simulink model "LowLevel_Example"  (R2024a)
settings: Solver=VariableStepAuto  StartTime=0.0  StopTime=10.0  RelTol=1e-3
model workspace (MAT data in the model file):
  Var = 0
  architecture_gsCommands = Simulink.Bus
  architecture_gsCommands.Alignment = -1
  architecture_gsCommands.PreserveElementDimensions = 0
  architecture_gsCommands.Elements_internal(1) = Simulink.BusElement
  architecture_gsCommands.Elements_internal(1).DimensionsMode = 'Fixed'
  architecture_gsCommands.Elements_internal(1).SamplingMode = 'Sample based'
  architecture_gsCommands.Elements_internal(1).SampleTime = -1
  architecture_gsCommands.Elements_internal(1).Name = 'apConfigParams'
  architecture_gsCommands.Elements_internal(1).DataType_internal = 'Bus: param_value_bus'
  architecture_gsCommands.Elements_internal(1).Complexity = 'real'
  architecture_gsCommands.Elements_internal(1).Dimensions = 1
  architecture_gsCommands.Elements_internal(2) = Simulink.BusElement
  architecture_gsCommands.Elements_internal(2).DimensionsMode = 'Fixed'
  architecture_gsCommands.Elements_internal(2).SamplingMode = 'Sample based'
  architecture_gsCommands.Elements_internal(2).SampleTime = -1
  architecture_gsCommands.Elements_internal(2).Name = 'gsCommands'
  architecture_gsCommands.Elements_internal(2).DataType_internal = 'Bus: gs_commands_bus'
  architecture_gsCommands.Elements_internal(2).Complexity = 'real'
  architecture_gsCommands.Elements_internal(2).Dimensions = 1
  architecture_gsCommands.Elements_internal(3) = Simulink.BusElement
  architecture_gsCommands.Elements_internal(3).DimensionsMode = 'Fixed'
  architecture_gsCommands.Elements_internal(3).SamplingMode = 'Sample based'
  architecture_gsCommands.Elements_internal(3).SampleTime = -1
  architecture_gsCommands.Elements_internal(3).Name = 'uavMission'
  architecture_gsCommands.Elements_internal(3).DataType_internal = 'Bus: mission_item_bus'
  architecture_gsCommands.Elements_internal(3).Complexity = 'real'
  architecture_gsCommands.Elements_internal(3).Dimensions = 1
  architecture_gsCommands.DataScope = 'Auto'
  ctrlSrfcDeflection = Simulink.Bus
  ctrlSrfcDeflection.Alignment = -1
  ctrlSrfcDeflection.PreserveElementDimensions = 0
  ctrlSrfcDeflection.Elements_internal(1) = Simulink.BusElement
  ctrlSrfcDeflection.Elements_internal(1).DimensionsMode = 'Fixed'
  ctrlSrfcDeflection.Elements_internal(1).SamplingMode = 'Sample based'
  ctrlSrfcDeflection.Elements_internal(1).SampleTime = -1
  ctrlSrfcDeflection.Elements_internal(1).Name = 'dA_dF'
  ctrlSrfcDeflection.Elements_internal(1).DataType_internal = 'double'
  ctrlSrfcDeflection.Elements_internal(1).Complexity = 'real'
  ctrlSrfcDeflection.Elements_internal(1).Dimensions = 1
  ctrlSrfcDeflection.Elements_internal(2) = Simulink.BusElement
  ctrlSrfcDeflection.Elements_internal(2).DimensionsMode = 'Fixed'
  ctrlSrfcDeflection.Elements_internal(2).SamplingMode = 'Sample based'
  ctrlSrfcDeflection.Elements_internal(2).SampleTime = -1
  ctrlSrfcDeflection.Elements_internal(2).Name = 'Brake'
  ctrlSrfcDeflection.Elements_internal(2).DataType_internal = 'double'
  ctrlSrfcDeflection.Elements_internal(2).Complexity = 'real'
  ctrlSrfcDeflection.Elements_internal(2).Dimensions = 1
  ctrlSrfcDeflection.Elements_internal(3) = Simulink.BusElement
  ctrlSrfcDeflection.Elements_internal(3).DimensionsMode = 'Fixed'
  ctrlSrfcDeflection.Elements_internal(3).SamplingMode = 'Sample based'
  ctrlSrfcDeflection.Elements_internal(3).SampleTime = -1
  ctrlSrfcDeflection.Elements_internal(3).Name = 'dR_dE'
  ctrlSrfcDeflection.Elements_internal(3).DataType_internal = 'double'
  ctrlSrfcDeflection.Elements_internal(3).Complexity = 'real'
  ctrlSrfcDeflection.Elements_internal(3).Dimensions = 1
  ctrlSrfcDeflection.DataScope = 'Auto'
  gs_commands_bus = Simulink.Bus
  gs_commands_bus.Alignment = -1
  gs_commands_bus.PreserveElementDimensions = 0
  gs_commands_bus.Elements_internal(1) = Simulink.BusElement
  gs_commands_bus.Elements_internal(1).DimensionsMode = 'Fixed'
  gs_commands_bus.Elements_internal(1).SamplingMode = 'Sample based'
  gs_commands_bus.Elements_internal(1).SampleTime = -1
  gs_commands_bus.Elements_internal(1).Description = 'Return to Base Command'
  gs_commands_bus.Elements_internal(1).Name = 'RTB'
  gs_commands_bus.Elements_internal(1).DataType_internal = 'uint8'
  gs_commands_bus.Elements_internal(1).Complexity = 'real'
  gs_commands_bus.Elements_internal(1).Dimensions = 1
  gs_commands_bus.Elements_internal(2) = Simulink.BusElement
  gs_commands_bus.Elements_internal(2).DimensionsMode = 'Fixed'
  gs_commands_bus.Elements_internal(2).SamplingMode = 'Sample based'
  gs_commands_bus.Elements_internal(2).SampleTime = -1
  gs_commands_bus.Elements_internal(2).Description = 'Airspeed Commanded by the GS'
  gs_commands_bus.Elements_internal(2).Name = 'U_c'
  gs_commands_bus.Elements_internal(2).DataType_internal = 'single'
  gs_commands_bus.Elements_internal(2).Complexity = 'real'
  gs_commands_bus.Elements_internal(2).Dimensions = 1
  gs_commands_bus.Elements_internal(3) = Simulink.BusElement
  gs_commands_bus.Elements_internal(3).DimensionsMode = 'Fixed'
  gs_commands_bus.Elements_internal(3).SamplingMode = 'Sample based'
  gs_commands_bus.Elements_internal(3).SampleTime = -1
  gs_commands_bus.Elements_internal(3).Description = 'Turnrate command when in mid Level Commands guidance mode'
  gs_commands_bus.Elements_internal(3).Name = 'psiDot_c_mdiLevel'
  gs_commands_bus.Elements_internal(3).DataType_internal = 'single'
  gs_commands_bus.Elements_internal(3).Complexity = 'real'
  gs_commands_bus.Elements_internal(3).Dimensions = 1
  gs_commands_bus.Elements_internal(4) = Simulink.BusElement
  gs_commands_bus.Elements_internal(4).DimensionsMode = 'Fixed'
  gs_commands_bus.Elements_internal(4).SamplingMode = 'Sample based'
  gs_commands_bus.Elements_internal(4).SampleTime = -1
  gs_commands_bus.Elements_internal(4).Description = 'Commanded altitude when in Mid Level Commands Mode. Also used as the altitude for RTB'
  gs_commands_bus.Elements_internal(4).Name = 'h_c_midLevel'
  gs_commands_bus.Elements_internal(4).DataType_internal = 'single'
  gs_commands_bus.Elements_internal(4).Complexity = 'real'
  gs_commands_bus.Elements_internal(4).Dimensions = 1
  gs_commands_bus.Elements_internal(5) = Simulink.BusElement
  gs_commands_bus.Elements_internal(5).DimensionsMode = 'Fixed'
  gs_commands_bus.Elements_internal(5).SamplingMode = 'Sample based'
  gs_commands_bus.Elements_internal(5).SampleTime = -1
  gs_commands_bus.Elements_internal(5).Name = 'isManualModeOn'
  gs_commands_bus.Elements_internal(5).DataType_internal = 'uint8'
  gs_commands_bus.Elements_internal(5).Complexity = 'real'
  gs_commands_bus.Elements_internal(5).Dimensions = 1
  gs_commands_bus.Elements_internal(6) = Simulink.BusElement
  gs_commands_bus.Elements_internal(6).DimensionsMode = 'Fixed'
  gs_commands_bus.Elements_internal(6).SamplingMode = 'Sample based'
  gs_commands_bus.Elements_internal(6).SampleTime = -1
  gs_commands_bus.Elements_internal(6).Name = 'viewPointIdx'
  gs_commands_bus.Elements_internal(6).DataType_internal = 'uint8'
  gs_commands_bus.Elements_internal(6).Complexity = 'real'
  gs_commands_bus.Elements_internal(6).Dimensions = 1
  gs_commands_bus.Elements_internal(7) = Simulink.BusElement
  gs_commands_bus.Elements_internal(7).DimensionsMode = 'Fixed'
  gs_commands_bus.Elements_internal(7).SamplingMode = 'Sample based'
  gs_commands_bus.Elements_internal(7).SampleTime = -1
  gs_commands_bus.Elements_internal(7).Name = 'guidanceMode'
  gs_commands_bus.Elements_internal(7).DataType_internal = 'uint8'
  gs_commands_bus.Elements_internal(7).Complexity = 'real'
  gs_commands_bus.Elements_internal(7).Dimensions = 1
  gs_commands_bus.DataScope = 'Auto'
  lightCmds = Simulink.Bus
  lightCmds.Alignment = -1
  lightCmds.PreserveElementDimensions = 0
  lightCmds.Elements_internal(1) = Simulink.BusElement
  lightCmds.Elements_internal(1).DimensionsMode = 'Fixed'
  lightCmds.Elements_internal(1).SamplingMode = 'Sample based'
  lightCmds.Elements_internal(1).SampleTime = -1
  lightCmds.Elements_internal(1).Name = 'NavigationLights'
  lightCmds.Elements_internal(1).DataType_internal = 'double'
  lightCmds.Elements_internal(1).Complexity = 'real'
  lightCmds.Elements_internal(1).Dimensions = 1
  lightCmds.Elements_internal(2) = Simulink.BusElement
  lightCmds.Elements_internal(2).DimensionsMode = 'Fixed'
  lightCmds.Elements_internal(2).SamplingMode = 'Sample based'
  lightCmds.Elements_internal(2).SampleTime = -1
  lightCmds.Elements_internal(2).Name = 'LandingStrobe'
  lightCmds.Elements_internal(2).DataType_internal = 'double'
  lightCmds.Elements_internal(2).Complexity = 'real'
  lightCmds.Elements_internal(2).Dimensions = 1
  lightCmds.DataScope = 'Auto'
  mission_item_bus = Simulink.Bus
  mission_item_bus.Alignment = -1
  mission_item_bus.PreserveElementDimensions = 0
  mission_item_bus.Elements_internal(1) = Simulink.BusElement
  mission_item_bus.Elements_internal(1).DimensionsMode = 'Fixed'
  mission_item_bus.Elements_internal(1).SamplingMode = 'Sample based'
  mission_item_bus.Elements_internal(1).SampleTime = -1
  mission_item_bus.Elements_internal(1).Description = 'PARAM1, see MAV_CMD enum'
  mission_item_bus.Elements_internal(1).Name = 'param1'
  mission_item_bus.Elements_internal(1).DataType_internal = 'single'
  mission_item_bus.Elements_internal(1).Complexity = 'real'
  mission_item_bus.Elements_internal(1).Dimensions = 1
  mission_item_bus.Elements_internal(2) = Simulink.BusElement
  mission_item_bus.Elements_internal(2).DimensionsMode = 'Fixed'
  mission_item_bus.Elements_internal(2).SamplingMode = 'Sample based'
  mission_item_bus.Elements_internal(2).SampleTime = -1
  mission_item_bus.Elements_internal(2).Description = 'PARAM4, see MAV_CMD enum'
  mission_item_bus.Elements_internal(2).Name = 'param4'
  mission_item_bus.Elements_internal(2).DataType_internal = 'single'
  mission_item_bus.Elements_internal(2).Complexity = 'real'
  mission_item_bus.Elements_internal(2).Dimensions = 1
  mission_item_bus.Elements_internal(3) = Simulink.BusElement
  mission_item_bus.Elements_internal(3).DimensionsMode = 'Fixed'
  mission_item_bus.Elements_internal(3).SamplingMode = 'Sample based'
  mission_item_bus.Elements_internal(3).SampleTime = -1
  mission_item_bus.Elements_internal(3).Description = 'PARAM3, see MAV_CMD enum'
  mission_item_bus.Elements_internal(3).Name = 'param3'
  mission_item_bus.Elements_internal(3).DataType_internal = 'single'
  mission_item_bus.Elements_internal(3).Complexity = 'real'
  mission_item_bus.Elements_internal(3).Dimensions = 1
  mission_item_bus.Elements_internal(4) = Simulink.BusElement
  mission_item_bus.Elements_internal(4).DimensionsMode = 'Fixed'
  mission_item_bus.Elements_internal(4).SamplingMode = 'Sample based'
  mission_item_bus.Elements_internal(4).SampleTime = -1
  mission_item_bus.Elements_internal(4).Description = 'false:0, true:1'
  mission_item_bus.Elements_internal(4).Name = 'current'
  mission_item_bus.Elements_internal(4).DataType_internal = 'uint8'
  mission_item_bus.Elements_internal(4).Complexity = 'real'
  mission_item_bus.Elements_internal(4).Dimensions = 1
  mission_item_bus.Elements_internal(5) = Simulink.BusElement
  mission_item_bus.Elements_internal(5).DimensionsMode = 'Fixed'
  mission_item_bus.Elements_internal(5).SamplingMode = 'Sample based'
  mission_item_bus.Elements_internal(5).SampleTime = -1
  mission_item_bus.Elements_internal(5).Description = 'PARAM2, see MAV_CMD enum'
  mission_item_bus.Elements_internal(5).Name = 'param2'
  mission_item_bus.Elements_internal(5).DataType_internal = 'single'
  mission_item_bus.Elements_internal(5).Complexity = 'real'
  mission_item_bus.Elements_internal(5).Dimensions = 1
  mission_item_bus.Elements_internal(6) = Simulink.BusElement
  mission_item_bus.Elements_internal(6).DimensionsMode = 'Fixed'
  mission_item_bus.Elements_internal(6).SamplingMode = 'Sample based'
  mission_item_bus.Elements_internal(6).SampleTime = -1
  mission_item_bus.Elements_internal(6).Description = 'PARAM5 / local: x position, global: latitude'
  mission_item_bus.Elements_internal(6).Name = 'x'
  mission_item_bus.Elements_internal(6).DataType_internal = 'single'
  mission_item_bus.Elements_internal(6).Complexity = 'real'
  mission_item_bus.Elements_internal(6).Dimensions = 1
  mission_item_bus.Elements_internal(7) = Simulink.BusElement
  mission_item_bus.Elements_internal(7).DimensionsMode = 'Fixed'
  mission_item_bus.Elements_internal(7).SamplingMode = 'Sample based'
  mission_item_bus.Elements_internal(7).SampleTime = -1
  mission_item_bus.Elements_internal(7).Description = 'PARAM6 / y position: global: longitude'
  mission_item_bus.Elements_internal(7).Name = 'y'
  mission_item_bus.Elements_internal(7).DataType_internal = 'single'
  mission_item_bus.Elements_internal(7).Complexity = 'real'
  mission_item_bus.Elements_internal(7).Dimensions = 1
  mission_item_bus.Elements_internal(8) = Simulink.BusElement
  mission_item_bus.Elements_internal(8).DimensionsMode = 'Fixed'
  mission_item_bus.Elements_internal(8).SamplingMode = 'Sample based'
  mission_item_bus.Elements_internal(8).SampleTime = -1
  mission_item_bus.Elements_internal(8).Description = 'The scheduled action for the waypoint. see MAV_CMD in common.xml MAVLink specs'
  mission_item_bus.Elements_internal(8).Name = 'command'
  mission_item_bus.Elements_internal(8).DataType_internal = 'uint16'
  mission_item_bus.Elements_internal(8).Complexity = 'real'
  mission_item_bus.Elements_internal(8).Dimensions = 1
  mission_item_bus.Elements_internal(9) = Simulink.BusElement
  mission_item_bus.Elements_internal(9).DimensionsMode = 'Fixed'
  mission_item_bus.Elements_internal(9).SamplingMode = 'Sample based'
  mission_item_bus.Elements_internal(9).SampleTime = -1
  mission_item_bus.Elements_internal(9).Description = 'PARAM7 / z position: global: altitude (relative or absolute, depending on frame.'
  mission_item_bus.Elements_internal(9).Name = 'z'
  mission_item_bus.Elements_internal(9).DataType_internal = 'single'
  mission_item_bus.Elements_internal(9).Complexity = 'real'
  mission_item_bus.Elements_internal(9).Dimensions = 1
  mission_item_bus.Elements_internal(10) = Simulink.BusElement
  mission_item_bus.Elements_internal(10).DimensionsMode = 'Fixed'
  mission_item_bus.Elements_internal(10).SamplingMode = 'Sample based'
  mission_item_bus.Elements_internal(10).SampleTime = -1
  mission_item_bus.Elements_internal(10).Description = 'System ID'
  mission_item_bus.Elements_internal(10).Name = 'target_system'
  mission_item_bus.Elements_internal(10).DataType_internal = 'uint8'
  mission_item_bus.Elements_internal(10).Complexity = 'real'
  mission_item_bus.Elements_internal(10).Dimensions = 1
  mission_item_bus.Elements_internal(11) = Simulink.BusElement
  mission_item_bus.Elements_internal(11).DimensionsMode = 'Fixed'
  mission_item_bus.Elements_internal(11).SamplingMode = 'Sample based'
  mission_item_bus.Elements_internal(11).SampleTime = -1
  mission_item_bus.Elements_internal(11).Description = 'Sequence'
  mission_item_bus.Elements_internal(11).Name = 'seq'
  mission_item_bus.Elements_internal(11).DataType_internal = 'uint16'
  mission_item_bus.Elements_internal(11).Complexity = 'real'
  mission_item_bus.Elements_internal(11).Dimensions = 1
  mission_item_bus.Elements_internal(12) = Simulink.BusElement
  mission_item_bus.Elements_internal(12).DimensionsMode = 'Fixed'
  mission_item_bus.Elements_internal(12).SamplingMode = 'Sample based'
  mission_item_bus.Elements_internal(12).SampleTime = -1
  mission_item_bus.Elements_internal(12).Description = 'Mission type, see MAV_MISSION_TYPE'
  mission_item_bus.Elements_internal(12).Name = 'mission_type'
  mission_item_bus.Elements_internal(12).DataType_internal = 'uint8'
  mission_item_bus.Elements_internal(12).Complexity = 'real'
  mission_item_bus.Elements_internal(12).Dimensions = 1
  mission_item_bus.Elements_internal(13) = Simulink.BusElement
  mission_item_bus.Elements_internal(13).DimensionsMode = 'Fixed'
  mission_item_bus.Elements_internal(13).SamplingMode = 'Sample based'
  mission_item_bus.Elements_internal(13).SampleTime = -1
  mission_item_bus.Elements_internal(13).Description = 'The coordinate system of the waypoint. see MAV_FRAME in mavlink_types.h'
  mission_item_bus.Elements_internal(13).Name = 'frame'
  mission_item_bus.Elements_internal(13).DataType_internal = 'uint8'
  mission_item_bus.Elements_internal(13).Complexity = 'real'
  mission_item_bus.Elements_internal(13).Dimensions = 1
  mission_item_bus.Elements_internal(14) = Simulink.BusElement
  mission_item_bus.Elements_internal(14).DimensionsMode = 'Fixed'
  mission_item_bus.Elements_internal(14).SamplingMode = 'Sample based'
  mission_item_bus.Elements_internal(14).SampleTime = -1
  mission_item_bus.Elements_internal(14).Description = 'Component ID'
  mission_item_bus.Elements_internal(14).Name = 'target_component'
  mission_item_bus.Elements_internal(14).DataType_internal = 'uint8'
  mission_item_bus.Elements_internal(14).Complexity = 'real'
  mission_item_bus.Elements_internal(14).Dimensions = 1
  mission_item_bus.Elements_internal(15) = Simulink.BusElement
  mission_item_bus.Elements_internal(15).DimensionsMode = 'Fixed'
  mission_item_bus.Elements_internal(15).SamplingMode = 'Sample based'
  mission_item_bus.Elements_internal(15).SampleTime = -1
  mission_item_bus.Elements_internal(15).Description = 'autocontinue to next wp'
  mission_item_bus.Elements_internal(15).Name = 'autocontinue'
  mission_item_bus.Elements_internal(15).DataType_internal = 'uint8'
  mission_item_bus.Elements_internal(15).Complexity = 'real'
  mission_item_bus.Elements_internal(15).Dimensions = 1
  mission_item_bus.DataScope = 'Auto'
  operatorCmds = Simulink.Bus
  operatorCmds.Alignment = -1
  operatorCmds.PreserveElementDimensions = 0
  operatorCmds.Elements_internal(1) = Simulink.BusElement
  operatorCmds.Elements_internal(1).DimensionsMode = 'Fixed'
  operatorCmds.Elements_internal(1).SamplingMode = 'Sample based'
  operatorCmds.Elements_internal(1).SampleTime = -1
  operatorCmds.Elements_internal(1).Name = 'RetractorCmds'
  operatorCmds.Elements_internal(1).DataType_internal = 'double'
  operatorCmds.Elements_internal(1).Complexity = 'real'
  operatorCmds.Elements_internal(1).Dimensions = 1
  operatorCmds.Elements_internal(2) = Simulink.BusElement
  operatorCmds.Elements_internal(2).DimensionsMode = 'Fixed'
  operatorCmds.Elements_internal(2).SamplingMode = 'Sample based'
  operatorCmds.Elements_internal(2).SampleTime = -1
  operatorCmds.Elements_internal(2).Name = 'PTZCmds'
  operatorCmds.Elements_internal(2).DataType_internal = 'double'
  operatorCmds.Elements_internal(2).Complexity = 'real'
  operatorCmds.Elements_internal(2).Dimensions = 1
  operatorCmds.DataScope = 'Auto'
  param_value_bus = Simulink.Bus
  param_value_bus.Alignment = -1
  param_value_bus.PreserveElementDimensions = 0
  param_value_bus.Elements_internal(1) = Simulink.BusElement
  param_value_bus.Elements_internal(1).DimensionsMode = 'Fixed'
  param_value_bus.Elements_internal(1).SamplingMode = 'Sample based'
  param_value_bus.Elements_internal(1).SampleTime = -1
  param_value_bus.Elements_internal(1).Description = 'Onboard parameter value'
  param_value_bus.Elements_internal(1).Name = 'param_value'
  param_value_bus.Elements_internal(1).DataType_internal = 'single'
  param_value_bus.Elements_internal(1).Complexity = 'real'
  param_value_bus.Elements_internal(1).Dimensions = 1
  param_value_bus.Elements_internal(2) = Simulink.BusElement
  param_value_bus.Elements_internal(2).DimensionsMode = 'Fixed'
  param_value_bus.Elements_internal(2).SamplingMode = 'Sample based'
  param_value_bus.Elements_internal(2).SampleTime = -1
  param_value_bus.Elements_internal(2).Description = 'Index of this onboard parameter'
  param_value_bus.Elements_internal(2).Name = 'param_index'
  param_value_bus.Elements_internal(2).DataType_internal = 'uint16'
  param_value_bus.Elements_internal(2).Complexity = 'real'
  param_value_bus.Elements_internal(2).Dimensions = 1
  param_value_bus.Elements_internal(3) = Simulink.BusElement
  param_value_bus.Elements_internal(3).DimensionsMode = 'Fixed'
  param_value_bus.Elements_internal(3).SamplingMode = 'Sample based'
  param_value_bus.Elements_internal(3).SampleTime = -1
  param_value_bus.Elements_internal(3).Description = 'Total number of onboard parameters'
  param_value_bus.Elements_internal(3).Name = 'param_count'
  param_value_bus.Elements_internal(3).DataType_internal = 'uint16'
  param_value_bus.Elements_internal(3).Complexity = 'real'
  param_value_bus.Elements_internal(3).Dimensions = 1
  param_value_bus.Elements_internal(4) = Simulink.BusElement
  param_value_bus.Elements_internal(4).DimensionsMode = 'Fixed'
  param_value_bus.Elements_internal(4).SamplingMode = 'Sample based'
  param_value_bus.Elements_internal(4).SampleTime = -1
  param_value_bus.Elements_internal(4).Description = 'Onboard parameter id, terminated by NULL if the length is less than 16 human-readable chars and WITHOUT null termination (NULL) byte if the length is exactly 16 chars - applications have to provide 16+1 bytes storage if the ID is stored as string'
  param_value_bus.Elements_internal(4).Name = 'param_id'
  param_value_bus.Elements_internal(4).DataType_internal = 'int8'
  param_value_bus.Elements_internal(4).Complexity = 'real'
  param_value_bus.Elements_internal(4).Dimensions = 16
  param_value_bus.Elements_internal(5) = Simulink.BusElement
  param_value_bus.Elements_internal(5).DimensionsMode = 'Fixed'
  param_value_bus.Elements_internal(5).SamplingMode = 'Sample based'
  param_value_bus.Elements_internal(5).SampleTime = -1
  param_value_bus.Elements_internal(5).Description = 'Onboard parameter type: see the MAV_PARAM_TYPE enum for supported data types.'
  param_value_bus.Elements_internal(5).Name = 'param_type'
  param_value_bus.Elements_internal(5).DataType_internal = 'uint8'
  param_value_bus.Elements_internal(5).Complexity = 'real'
  param_value_bus.Elements_internal(5).Dimensions = 1
  param_value_bus.DataScope = 'Auto'
(part 1 of 2)
settings Model: Creator=The MathWorks, Inc.  LastModifiedBy=Tamir Azaouag
settings SolverCC: AlgebraicLoopSolver=TrustRegion
settings DebuggingCC: UnconnectedLineMsg=warning
settings ModelReferenceCC: EnableRefExpFcnMdlSchedulingChecks=on
settings RTWCC: GPUComputeCapability=3.5  DLArmComputeVersion=19.05

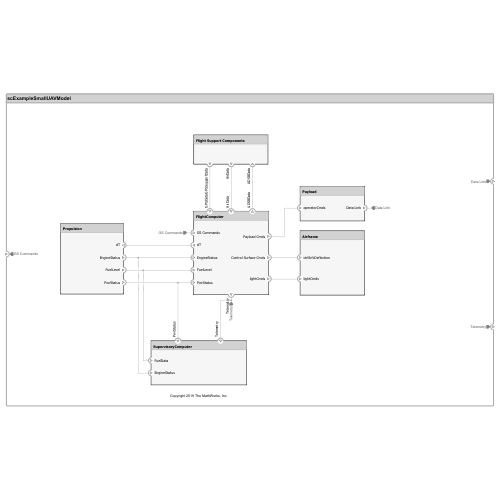
[thumbnail: Simulink's stored preview of the top-level diagram]
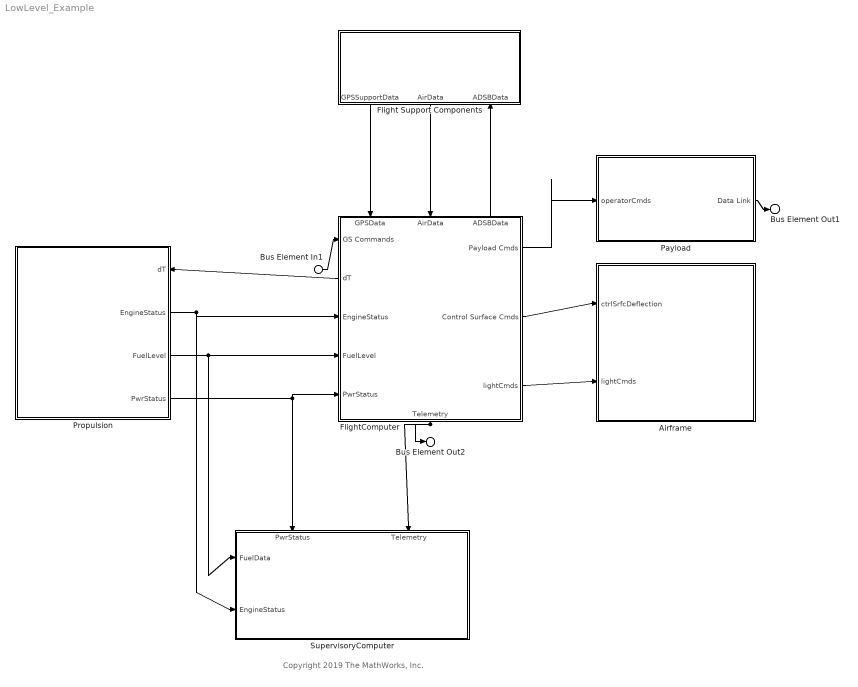
== system LowLevel_Example ==
  note: Copyright 2019 The MathWorks, Inc.
  Bus Element In1 : Inport  PortName=GS Commands
  Airframe : Subsystem
      settings: PortSchema="{\"entries\":[{\"content\":{\"headerSize\":26,\"margin\":15,\"minimumSpacing\":25,\"sides\":[{\"content\":{\"connectorIds\":[\"In1\",\"In2\"]},\"type\":\"ConnectorPlacement.EquallySpacedRectSide\",\"uuid\":\"410c5b0f-08b5-48c1-aeab-ad32707f18cb\"},{\"content\":{\"connectorIds\":[],\"side\":\"RIGHT\"},\"type\":\"ConnectorPlacement.EquallySpacedRectSide\",\"uuid\":\"175f376c-06cb-43d8-93cf-cfe74288c6ca\"},{\"content\":{\"connectorIds\":[],\"side\":\"TOP\"},\"type\":\"ConnectorPlacement.EquallySpacedRectSide\",\"uuid\":\"49daa1ce-2b00-43ab-833d-e4aa679275fe\"}]},\"type\":\"ConnectorPlacement.EquallySpacedConnector\",\"uuid\":\"5fe6ec80-a25e-4dcf-8012-d525fb653d3d\"}],\"packageUris\":[\"http:\\/\\/schema.mathworks.com\\/mf0\\/Connector\\/19700101\"],\"version\":\"1.0\"}"
  Flight Support Components : Subsystem
      settings: PortSchema="{\"entries\":[{\"content\":{\"headerSize\":26,\"margin\":15,\"minimumSpacing\":25,\"sides\":[{\"content\":{\"connectorIds\":[]},\"type\":\"ConnectorPlacement.EquallySpacedRectSide\",\"uuid\":\"410c5b0f-08b5-48c1-aeab-ad32707f18cb\"},{\"content\":{\"connectorIds\":[],\"side\":\"RIGHT\"},\"type\":\"ConnectorPlacement.EquallySpacedRectSide\",\"uuid\":\"175f376c-06cb-43d8-93cf-cfe74288c6ca\"},{\"content\":{\"connectorIds\":[],\"side\":\"TOP\"},\"type\":\"ConnectorPlacement.EquallySpacedRectSide\",\"uuid\":\"49daa1ce-2b00-43ab-833d-e4aa679275fe\"},{\"content\":{\"connectorIds\":[\"Out2\",\"Out1\",\"In1\"],\"side\":\"BOTTOM\"},\"type\":\"ConnectorPlacement.EquallySpacedRectSide\",\"uuid\":\"223cc250-646f-4cb8-9a9a-650b4875d99e\"}]},\"type\":\"ConnectorPlacement.EquallySpacedConnector\",\"uuid\":\"5fe6ec80-a25e-4dcf-8012-d525fb653d3d\"}],\"packageUris\":[\"http:\\/\\/schema.mathworks.com\\/mf0\\/Connector\\/19700101\"],\"version\":\"1.0\"}"
  FlightComputer : Subsystem
      settings: PortSchema="{\"entries\":[{\"content\":{\"headerSize\":26,\"margin\":15,\"minimumSpacing\":25,\"sides\":[{\"content\":{\"connectorIds\":[\"In5\",\"Out5\",\"In2\",\"In3\",\"In6\"]},\"type\":\"ConnectorPlacement.EquallySpacedRectSide\",\"uuid\":\"288187f8-f80a-4535-8eff-6998f4e932c0\"},{\"content\":{\"connectorIds\":[\"Out3\",\"Out2\",\"Out6\"],\"side\":\"RIGHT\"},\"type\":\"ConnectorPlacement.EquallySpacedRectSide\",\"uuid\":\"d1e22774-cdd2-4e71-94b1-3e938d9d16f6\"},{\"content\":{\"connectorIds\":[\"In4\",\"In1\",\"Out1\"],\"side\":\"TOP\"},\"type\":\"ConnectorPlacement.EquallySpacedRectSide\",\"uuid\":\"890411bd-a9cd-40b1-a683-0574f0cd14d7\"},{\"content\":{\"connectorIds\":[\"Out4\"],\"side\":\"BOTTOM\"},\"type\":\"ConnectorPlacement.EquallySpacedRectSide\",\"uuid\":\"5b2b87a3-00cb-493f-9187-a9231b1dbd9e\"}]},\"type\":\"ConnectorPlacement.EquallySpacedConnector\",\"uuid\":\"f677e6f7-ddb0-43ad-ab3a-7892dac74d79\"}],\"packageUris\":[\"http:\\/\\/schema.mathworks.com\\/mf0\\/Connector\\/19700101\"],\"version\":\"1.0\"}"
  Payload : Subsystem
      settings: PortSchema="{\"entries\":[{\"content\":{\"headerSize\":26,\"margin\":15,\"minimumSpacing\":25,\"sides\":[{\"content\":{\"connectorIds\":[\"In1\"]},\"type\":\"ConnectorPlacement.EquallySpacedRectSide\",\"uuid\":\"288187f8-f80a-4535-8eff-6998f4e932c0\"},{\"content\":{\"connectorIds\":[\"Out1\"],\"side\":\"RIGHT\"},\"type\":\"ConnectorPlacement.EquallySpacedRectSide\",\"uuid\":\"d1e22774-cdd2-4e71-94b1-3e938d9d16f6\"},{\"content\":{\"connectorIds\":[],\"side\":\"TOP\"},\"type\":\"ConnectorPlacement.EquallySpacedRectSide\",\"uuid\":\"890411bd-a9cd-40b1-a683-0574f0cd14d7\"}]},\"type\":\"ConnectorPlacement.EquallySpacedConnector\",\"uuid\":\"f677e6f7-ddb0-43ad-ab3a-7892dac74d79\"}],\"packageUris\":[\"http:\\/\\/schema.mathworks.com\\/mf0\\/Connector\\/19700101\"],\"version\":\"1.0\"}"
  Propulsion : Subsystem
      settings: PortSchema="{\"entries\":[{\"content\":{\"headerSize\":26,\"margin\":15,\"minimumSpacing\":25,\"sides\":[{\"content\":{\"connectorIds\":[]},\"type\":\"ConnectorPlacement.EquallySpacedRectSide\",\"uuid\":\"288187f8-f80a-4535-8eff-6998f4e932c0\"},{\"content\":{\"connectorIds\":[\"In1\",\"Out1\",\"Out2\",\"Out3\"],\"side\":\"RIGHT\"},\"type\":\"ConnectorPlacement.EquallySpacedRectSide\",\"uuid\":\"d1e22774-cdd2-4e71-94b1-3e938d9d16f6\"},{\"content\":{\"connectorIds\":[],\"side\":\"TOP\"},\"type\":\"ConnectorPlacement.EquallySpacedRectSide\",\"uuid\":\"890411bd-a9cd-40b1-a683-0574f0cd14d7\"}]},\"type\":\"ConnectorPlacement.EquallySpacedConnector\",\"uuid\":\"f677e6f7-ddb0-43ad-ab3a-7892dac74d79\"}],\"packageUris\":[\"http:\\/\\/schema.mathworks.com\\/mf0\\/Connector\\/19700101\"],\"version\":\"1.0\"}"
  SupervisoryComputer : Subsystem
      settings: PortSchema="{\"entries\":[{\"content\":{\"headerSize\":26,\"margin\":15,\"minimumSpacing\":25,\"sides\":[{\"content\":{\"connectorIds\":[\"In2\",\"In1\"]},\"type\":\"ConnectorPlacement.EquallySpacedRectSide\",\"uuid\":\"410c5b0f-08b5-48c1-aeab-ad32707f18cb\"},{\"content\":{\"connectorIds\":[],\"side\":\"RIGHT\"},\"type\":\"ConnectorPlacement.EquallySpacedRectSide\",\"uuid\":\"175f376c-06cb-43d8-93cf-cfe74288c6ca\"},{\"content\":{\"connectorIds\":[\"In3\",\"In4\"],\"side\":\"TOP\"},\"type\":\"ConnectorPlacement.EquallySpacedRectSide\",\"uuid\":\"49daa1ce-2b00-43ab-833d-e4aa679275fe\"}]},\"type\":\"ConnectorPlacement.EquallySpacedConnector\",\"uuid\":\"5fe6ec80-a25e-4dcf-8012-d525fb653d3d\"}],\"packageUris\":[\"http:\\/\\/schema.mathworks.com\\/mf0\\/Connector\\/19700101\"],\"version\":\"1.0\"}"
  Bus Element Out1 : Outport  VectorParamsAs1DForOutWhenUnconnected=off  PortName=Data Link
  Bus Element Out2 : Outport  Port=2  VectorParamsAs1DForOutWhenUnconnected=off  PortName=Telemetry
  wires:
  FlightComputer/1(ADSBData) -> Flight Support Components/1(ADSBData)
  FlightComputer/6(lightCmds) -> Airframe/2(lightCmds)
  Flight Support Components/1(AirData) -> FlightComputer/1(AirData)
  FlightComputer/2(Control Surface Cmds) -> Airframe/1(ctrlSrfcDeflection)
  Flight Support Components/2(GPSSupportData) -> FlightComputer/4(GPSData)
  FlightComputer/5(dT) -> Propulsion/1(dT)
  Payload/1(Data Link) -> Bus Element Out1/1
  FlightComputer/4(Telemetry) -> SupervisoryComputer/4(Telemetry), Bus Element Out2/1
  FlightComputer/3(Payload Cmds) -> Payload/1(operatorCmds)
  Bus Element In1/1 -> FlightComputer/5(GS Commands)
  Propulsion/2(FuelLevel) -> FlightComputer/3(FuelLevel), SupervisoryComputer/2(FuelData)
  Propulsion/3(PwrStatus) -> FlightComputer/6(PwrStatus), SupervisoryComputer/3(PwrStatus)
  Propulsion/1(EngineStatus) -> SupervisoryComputer/1(EngineStatus), FlightComputer/2(EngineStatus)

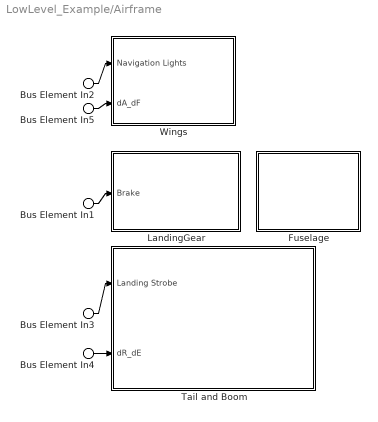
== system LowLevel_Example/Airframe ==
  Bus Element In5 : Inport  PortName=ctrlSrfcDeflection  Element=dA_dF
  Bus Element In1 : Inport  PortName=ctrlSrfcDeflection  Element=Brake
  Bus Element In4 : Inport  PortName=ctrlSrfcDeflection  Element=dR_dE
  Bus Element In2 : Inport  Port=2  PortName=lightCmds  Element=NavigationLights
  Bus Element In3 : Inport  Port=2  PortName=lightCmds  Element=LandingStrobe
  Fuselage : Subsystem
      settings: PortSchema="{\"entries\":[{\"content\":{\"headerSize\":26,\"margin\":15,\"minimumSpacing\":25,\"sides\":[{\"content\":{\"connectorIds\":[]},\"type\":\"ConnectorPlacement.EquallySpacedRectSide\",\"uuid\":\"1d3f3a23-636b-441d-85a6-b75e05b18389\"},{\"content\":{\"connectorIds\":[],\"side\":\"RIGHT\"},\"type\":\"ConnectorPlacement.EquallySpacedRectSide\",\"uuid\":\"e22d7e46-f58c-4c9d-8892-998381cd60e3\"},{\"content\":{\"connectorIds\":[],\"side\":\"TOP\"},\"type\":\"ConnectorPlacement.EquallySpacedRectSide\",\"uuid\":\"8b16ddbb-b471-4974-8372-55ce1efe9f0b\"}]},\"type\":\"ConnectorPlacement.EquallySpacedConnector\",\"uuid\":\"3aaecc83-0a24-4c0b-b096-52d61c24d002\"}],\"packageUris\":[\"http:\\/\\/schema.mathworks.com\\/mf0\\/Connector\\/19700101\"],\"version\":\"1.0\"}"
  LandingGear : Subsystem
      settings: PortSchema="{\"entries\":[{\"content\":{\"headerSize\":26,\"margin\":15,\"minimumSpacing\":25,\"sides\":[{\"content\":{\"connectorIds\":[\"In1\"]},\"type\":\"ConnectorPlacement.EquallySpacedRectSide\",\"uuid\":\"410c5b0f-08b5-48c1-aeab-ad32707f18cb\"},{\"content\":{\"connectorIds\":[],\"side\":\"RIGHT\"},\"type\":\"ConnectorPlacement.EquallySpacedRectSide\",\"uuid\":\"175f376c-06cb-43d8-93cf-cfe74288c6ca\"},{\"content\":{\"connectorIds\":[],\"side\":\"TOP\"},\"type\":\"ConnectorPlacement.EquallySpacedRectSide\",\"uuid\":\"49daa1ce-2b00-43ab-833d-e4aa679275fe\"}]},\"type\":\"ConnectorPlacement.EquallySpacedConnector\",\"uuid\":\"5fe6ec80-a25e-4dcf-8012-d525fb653d3d\"}],\"packageUris\":[\"http:\\/\\/schema.mathworks.com\\/mf0\\/Connector\\/19700101\"],\"version\":\"1.0\"}"
  Tail and Boom : Subsystem
      settings: PortSchema="{\"entries\":[{\"content\":{\"headerSize\":26,\"margin\":15,\"minimumSpacing\":25,\"sides\":[{\"content\":{\"connectorIds\":[\"In1\",\"In2\"]},\"type\":\"ConnectorPlacement.EquallySpacedRectSide\",\"uuid\":\"410c5b0f-08b5-48c1-aeab-ad32707f18cb\"},{\"content\":{\"connectorIds\":[],\"side\":\"RIGHT\"},\"type\":\"ConnectorPlacement.EquallySpacedRectSide\",\"uuid\":\"175f376c-06cb-43d8-93cf-cfe74288c6ca\"},{\"content\":{\"connectorIds\":[],\"side\":\"TOP\"},\"type\":\"ConnectorPlacement.EquallySpacedRectSide\",\"uuid\":\"49daa1ce-2b00-43ab-833d-e4aa679275fe\"}]},\"type\":\"ConnectorPlacement.EquallySpacedConnector\",\"uuid\":\"5fe6ec80-a25e-4dcf-8012-d525fb653d3d\"}],\"packageUris\":[\"http:\\/\\/schema.mathworks.com\\/mf0\\/Connector\\/19700101\"],\"version\":\"1.0\"}"
  Wings : Subsystem
      settings: PortSchema="{\"entries\":[{\"content\":{\"headerSize\":26,\"margin\":15,\"minimumSpacing\":25,\"sides\":[{\"content\":{\"connectorIds\":[\"In1\",\"In2\"]},\"type\":\"ConnectorPlacement.EquallySpacedRectSide\",\"uuid\":\"410c5b0f-08b5-48c1-aeab-ad32707f18cb\"},{\"content\":{\"connectorIds\":[],\"side\":\"RIGHT\"},\"type\":\"ConnectorPlacement.EquallySpacedRectSide\",\"uuid\":\"175f376c-06cb-43d8-93cf-cfe74288c6ca\"},{\"content\":{\"connectorIds\":[],\"side\":\"TOP\"},\"type\":\"ConnectorPlacement.EquallySpacedRectSide\",\"uuid\":\"49daa1ce-2b00-43ab-833d-e4aa679275fe\"}]},\"type\":\"ConnectorPlacement.EquallySpacedConnector\",\"uuid\":\"5fe6ec80-a25e-4dcf-8012-d525fb653d3d\"}],\"packageUris\":[\"http:\\/\\/schema.mathworks.com\\/mf0\\/Connector\\/19700101\"],\"version\":\"1.0\"}"
  wires:
  Bus Element In2/1 -> Wings/1(Navigation Lights)
  Bus Element In3/1 -> Tail and Boom/1(Landing Strobe)
  Bus Element In5/1 -> Wings/2(dA_dF)
  Bus Element In1/1 -> LandingGear/1(Brake)
  Bus Element In4/1 -> Tail and Boom/2(dR_dE)

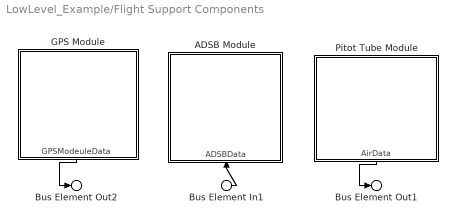
== system LowLevel_Example/Flight Support Components ==
  Bus Element In1 : Inport  PortName=ADSBData
  ADSB Module : Subsystem
      settings: PortSchema="{\"entries\":[{\"content\":{\"headerSize\":26,\"margin\":15,\"minimumSpacing\":25,\"sides\":[{\"content\":{\"connectorIds\":[]},\"type\":\"ConnectorPlacement.EquallySpacedRectSide\",\"uuid\":\"d72055ff-278e-465f-ba3e-c6c3db7bfef8\"},{\"content\":{\"connectorIds\":[],\"side\":\"RIGHT\"},\"type\":\"ConnectorPlacement.EquallySpacedRectSide\",\"uuid\":\"8524ed89-5b6f-4252-b4a0-99bfa4432df7\"},{\"content\":{\"connectorIds\":[],\"side\":\"TOP\"},\"type\":\"ConnectorPlacement.EquallySpacedRectSide\",\"uuid\":\"146bf699-8817-45e5-9f2f-d03ccee27e91\"},{\"content\":{\"connectorIds\":[\"In1\"],\"side\":\"BOTTOM\"},\"type\":\"ConnectorPlacement.EquallySpacedRectSide\",\"uuid\":\"d98fe66c-9b12-4e8f-882a-fe3e8718818f\"}]},\"type\":\"ConnectorPlacement.EquallySpacedConnector\",\"uuid\":\"07a8b4ff-7c12-4fb8-a327-ae9aaef314be\"}],\"packageUris\":[\"http:\\/\\/schema.mathworks.com\\/mf0\\/Connector\\/19700101\"],\"version\":\"1.0\"}"
  GPS Module : Subsystem
      settings: PortSchema="{\"entries\":[{\"content\":{\"headerSize\":26,\"margin\":15,\"minimumSpacing\":25,\"sides\":[{\"content\":{\"connectorIds\":[]},\"type\":\"ConnectorPlacement.EquallySpacedRectSide\",\"uuid\":\"9f35dc00-989c-4612-aee9-27ffd041f5d2\"},{\"content\":{\"connectorIds\":[],\"side\":\"RIGHT\"},\"type\":\"ConnectorPlacement.EquallySpacedRectSide\",\"uuid\":\"fc636a36-c80d-4d26-be49-cb148246bb8f\"},{\"content\":{\"connectorIds\":[],\"side\":\"TOP\"},\"type\":\"ConnectorPlacement.EquallySpacedRectSide\",\"uuid\":\"9fe3dfb0-e690-4d7f-8c9a-5f9d40a5a564\"},{\"content\":{\"connectorIds\":[\"Out1\"],\"side\":\"BOTTOM\"},\"type\":\"ConnectorPlacement.EquallySpacedRectSide\",\"uuid\":\"849be294-e2a5-439f-8ad2-64d927b9f694\"}]},\"type\":\"ConnectorPlacement.EquallySpacedConnector\",\"uuid\":\"46c87048-a43e-442c-ad6b-39b68668708d\"}],\"packageUris\":[\"http:\\/\\/schema.mathworks.com\\/mf0\\/Connector\\/19700101\"],\"version\":\"1.0\"}"
  Pitot Tube Module : Subsystem
      settings: PortSchema="{\"entries\":[{\"content\":{\"headerSize\":26,\"margin\":15,\"minimumSpacing\":25,\"sides\":[{\"content\":{\"connectorIds\":[]},\"type\":\"ConnectorPlacement.EquallySpacedRectSide\",\"uuid\":\"288187f8-f80a-4535-8eff-6998f4e932c0\"},{\"content\":{\"connectorIds\":[],\"side\":\"RIGHT\"},\"type\":\"ConnectorPlacement.EquallySpacedRectSide\",\"uuid\":\"d1e22774-cdd2-4e71-94b1-3e938d9d16f6\"},{\"content\":{\"connectorIds\":[],\"side\":\"TOP\"},\"type\":\"ConnectorPlacement.EquallySpacedRectSide\",\"uuid\":\"890411bd-a9cd-40b1-a683-0574f0cd14d7\"},{\"content\":{\"connectorIds\":[\"Out1\"],\"side\":\"BOTTOM\"},\"type\":\"ConnectorPlacement.EquallySpacedRectSide\",\"uuid\":\"13559410-32ac-48b6-8b1d-f616ead46f43\"}]},\"type\":\"ConnectorPlacement.EquallySpacedConnector\",\"uuid\":\"f677e6f7-ddb0-43ad-ab3a-7892dac74d79\"}],\"packageUris\":[\"http:\\/\\/schema.mathworks.com\\/mf0\\/Connector\\/19700101\"],\"version\":\"1.0\"}"
  Bus Element Out1 : Outport  VectorParamsAs1DForOutWhenUnconnected=off  PortName=AirData
  Bus Element Out2 : Outport  Port=2  VectorParamsAs1DForOutWhenUnconnected=off  PortName=GPSSupportData
  wires:
  Pitot Tube Module/1(AirData) -> Bus Element Out1/1
  GPS Module/1(GPSModeuleData) -> Bus Element Out2/1
  Bus Element In1/1 -> ADSB Module/1(ADSBData)

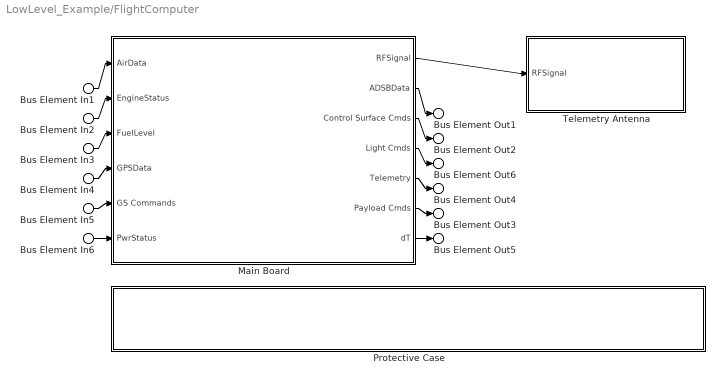
== system LowLevel_Example/FlightComputer ==
  Bus Element In1 : Inport  PortName=AirData
  Bus Element In2 : Inport  Port=2  PortName=EngineStatus
  Bus Element In3 : Inport  Port=3  PortName=FuelLevel
  Bus Element In4 : Inport  Port=4  PortName=GPSData
  Bus Element In5 : Inport  Port=5  PortName=GS Commands
  Bus Element In6 : Inport  Port=6  PortName=PwrStatus
  Main Board : Subsystem
      settings: PortSchema="{\"entries\":[{\"content\":{\"headerSize\":26,\"margin\":15,\"minimumSpacing\":25,\"sides\":[{\"content\":{\"connectorIds\":[\"In1\",\"In2\",\"In3\",\"In4\",\"In5\",\"In6\"]},\"type\":\"ConnectorPlacement.EquallySpacedRectSide\",\"uuid\":\"288187f8-f80a-4535-8eff-6998f4e932c0\"},{\"content\":{\"connectorIds\":[\"Out1\",\"Out2\",\"Out3\",\"Out4\",\"Out5\",\"Out6\",\"Out7\"],\"side\":\"RIGHT\"},\"type\":\"ConnectorPlacement.EquallySpacedRectSide\",\"uuid\":\"d1e22774-cdd2-4e71-94b1-3e938d9d16f6\"},{\"content\":{\"connectorIds\":[],\"side\":\"TOP\"},\"type\":\"ConnectorPlacement.EquallySpacedRectSide\",\"uuid\":\"890411bd-a9cd-40b1-a683-0574f0cd14d7\"}]},\"type\":\"ConnectorPlacement.EquallySpacedConnector\",\"uuid\":\"f677e6f7-ddb0-43ad-ab3a-7892dac74d79\"}],\"packageUris\":[\"http:\\/\\/schema.mathworks.com\\/mf0\\/Connector\\/19700101\"],\"version\":\"1.0\"}"
  Protective Case : Subsystem
      settings: PortSchema="{\"entries\":[{\"content\":{\"headerSize\":26,\"margin\":15,\"minimumSpacing\":25,\"sides\":[{\"content\":{\"connectorIds\":[]},\"type\":\"ConnectorPlacement.EquallySpacedRectSide\",\"uuid\":\"1d3f3a23-636b-441d-85a6-b75e05b18389\"},{\"content\":{\"connectorIds\":[],\"side\":\"RIGHT\"},\"type\":\"ConnectorPlacement.EquallySpacedRectSide\",\"uuid\":\"e22d7e46-f58c-4c9d-8892-998381cd60e3\"},{\"content\":{\"connectorIds\":[],\"side\":\"TOP\"},\"type\":\"ConnectorPlacement.EquallySpacedRectSide\",\"uuid\":\"8b16ddbb-b471-4974-8372-55ce1efe9f0b\"}]},\"type\":\"ConnectorPlacement.EquallySpacedConnector\",\"uuid\":\"3aaecc83-0a24-4c0b-b096-52d61c24d002\"}],\"packageUris\":[\"http:\\/\\/schema.mathworks.com\\/mf0\\/Connector\\/19700101\"],\"version\":\"1.0\"}"
  Telemetry Antenna : Subsystem
      settings: PortSchema="{\"entries\":[{\"content\":{\"headerSize\":26,\"margin\":15,\"minimumSpacing\":25,\"sides\":[{\"content\":{\"connectorIds\":[\"In1\"]},\"type\":\"ConnectorPlacement.EquallySpacedRectSide\",\"uuid\":\"1d3f3a23-636b-441d-85a6-b75e05b18389\"},{\"content\":{\"connectorIds\":[],\"side\":\"RIGHT\"},\"type\":\"ConnectorPlacement.EquallySpacedRectSide\",\"uuid\":\"e22d7e46-f58c-4c9d-8892-998381cd60e3\"},{\"content\":{\"connectorIds\":[],\"side\":\"TOP\"},\"type\":\"ConnectorPlacement.EquallySpacedRectSide\",\"uuid\":\"8b16ddbb-b471-4974-8372-55ce1efe9f0b\"}]},\"type\":\"ConnectorPlacement.EquallySpacedConnector\",\"uuid\":\"3aaecc83-0a24-4c0b-b096-52d61c24d002\"}],\"packageUris\":[\"http:\\/\\/schema.mathworks.com\\/mf0\\/Connector\\/19700101\"],\"version\":\"1.0\"}"
  Bus Element Out1 : Outport  VectorParamsAs1DForOutWhenUnconnected=off  PortName=ADSBData
  Bus Element Out2 : Outport  Port=2  VectorParamsAs1DForOutWhenUnconnected=off  PortName=Control Surface Cmds
  Bus Element Out3 : Outport  Port=3  VectorParamsAs1DForOutWhenUnconnected=off  PortName=Payload Cmds
  Bus Element Out4 : Outport  Port=4  VectorParamsAs1DForOutWhenUnconnected=off  PortName=Telemetry
  Bus Element Out5 : Outport  Port=5  VectorParamsAs1DForOutWhenUnconnected=off  PortName=dT
  Bus Element Out6 : Outport  Port=6  VectorParamsAs1DForOutWhenUnconnected=off  PortName=lightCmds
  wires:
  Bus Element In4/1 -> Main Board/4(GPSData)
  Bus Element In1/1 -> Main Board/1(AirData)
  Main Board/2(ADSBData) -> Bus Element Out1/1
  Bus Element In2/1 -> Main Board/2(EngineStatus)
  Main Board/5(Telemetry) -> Bus Element Out4/1
  Main Board/4(Light Cmds) -> Bus Element Out6/1
  Bus Element In3/1 -> Main Board/3(FuelLevel)
  Bus Element In6/1 -> Main Board/6(PwrStatus)
  Bus Element In5/1 -> Main Board/5(GS Commands)
  Main Board/3(Control Surface Cmds) -> Bus Element Out2/1
  Main Board/6(Payload Cmds) -> Bus Element Out3/1
  Main Board/7(dT) -> Bus Element Out5/1
  Main Board/1(RFSignal) -> Telemetry Antenna/1(RFSignal)

== system LowLevel_Example/Payload ==
  Bus Element In1 : Inport  PortName=operatorCmds
  Payload : Subsystem
      settings: PortSchema="{\"entries\":[{\"content\":{\"headerSize\":26,\"margin\":15,\"minimumSpacing\":25,\"sides\":[{\"content\":{\"connectorIds\":[\"In1\"]},\"type\":\"ConnectorPlacement.EquallySpacedRectSide\",\"uuid\":\"288187f8-f80a-4535-8eff-6998f4e932c0\"},{\"content\":{\"connectorIds\":[\"Out1\"],\"side\":\"RIGHT\"},\"type\":\"ConnectorPlacement.EquallySpacedRectSide\",\"uuid\":\"d1e22774-cdd2-4e71-94b1-3e938d9d16f6\"},{\"content\":{\"connectorIds\":[],\"side\":\"TOP\"},\"type\":\"ConnectorPlacement.EquallySpacedRectSide\",\"uuid\":\"890411bd-a9cd-40b1-a683-0574f0cd14d7\"}]},\"type\":\"ConnectorPlacement.EquallySpacedConnector\",\"uuid\":\"f677e6f7-ddb0-43ad-ab3a-7892dac74d79\"}],\"packageUris\":[\"http:\\/\\/schema.mathworks.com\\/mf0\\/Connector\\/19700101\"],\"version\":\"1.0\"}"
  Payload Data Link : Subsystem
      settings: PortSchema="{\"entries\":[{\"content\":{\"headerSize\":26,\"margin\":15,\"minimumSpacing\":25,\"sides\":[{\"content\":{\"connectorIds\":[\"In1\"]},\"type\":\"ConnectorPlacement.EquallySpacedRectSide\",\"uuid\":\"288187f8-f80a-4535-8eff-6998f4e932c0\"},{\"content\":{\"connectorIds\":[\"Out1\"],\"side\":\"RIGHT\"},\"type\":\"ConnectorPlacement.EquallySpacedRectSide\",\"uuid\":\"d1e22774-cdd2-4e71-94b1-3e938d9d16f6\"},{\"content\":{\"connectorIds\":[],\"side\":\"TOP\"},\"type\":\"ConnectorPlacement.EquallySpacedRectSide\",\"uuid\":\"890411bd-a9cd-40b1-a683-0574f0cd14d7\"}]},\"type\":\"ConnectorPlacement.EquallySpacedConnector\",\"uuid\":\"f677e6f7-ddb0-43ad-ab3a-7892dac74d79\"}],\"packageUris\":[\"http:\\/\\/schema.mathworks.com\\/mf0\\/Connector\\/19700101\"],\"version\":\"1.0\"}"
  Bus Element Out1 : Outport  VectorParamsAs1DForOutWhenUnconnected=off  PortName=Data Link
  wires:
  Bus Element In1/1 -> Payload/1(operatorCmds)
  Payload/1(Video Out) -> Payload Data Link/1(Video In)
  Payload Data Link/1(Data Link) -> Bus Element Out1/1

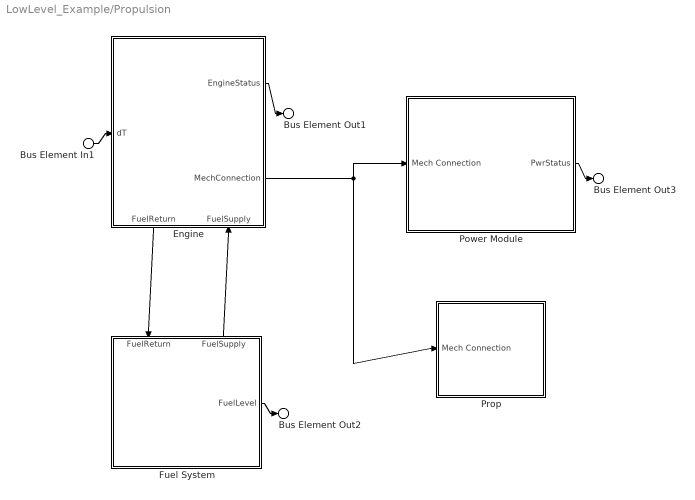
== system LowLevel_Example/Propulsion ==
  Bus Element In1 : Inport  PortName=dT
  Engine : Subsystem
      settings: PortSchema="{\"entries\":[{\"content\":{\"headerSize\":26,\"margin\":15,\"minimumSpacing\":25,\"sides\":[{\"content\":{\"connectorIds\":[\"In2\"]},\"type\":\"ConnectorPlacement.EquallySpacedRectSide\",\"uuid\":\"288187f8-f80a-4535-8eff-6998f4e932c0\"},{\"content\":{\"connectorIds\":[\"Out1\",\"Out3\"],\"side\":\"RIGHT\"},\"type\":\"ConnectorPlacement.EquallySpacedRectSide\",\"uuid\":\"d1e22774-cdd2-4e71-94b1-3e938d9d16f6\"},{\"content\":{\"connectorIds\":[],\"side\":\"TOP\"},\"type\":\"ConnectorPlacement.EquallySpacedRectSide\",\"uuid\":\"890411bd-a9cd-40b1-a683-0574f0cd14d7\"},{\"content\":{\"connectorIds\":[\"Out2\",\"In1\"],\"side\":\"BOTTOM\"},\"type\":\"ConnectorPlacement.EquallySpacedRectSide\",\"uuid\":\"cb804324-7012-4a66-9d89-240ca07e311a\"}]},\"type\":\"ConnectorPlacement.EquallySpacedConnector\",\"uuid\":\"f677e6f7-ddb0-43ad-ab3a-7892dac74d79\"}],\"packageUris\":[\"http:\\/\\/schema.mathworks.com\\/mf0\\/Connector\\/19700101\"],\"version\":\"1.0\"}"
  Fuel System : Subsystem
      settings: PortSchema="{\"entries\":[{\"content\":{\"headerSize\":26,\"margin\":15,\"minimumSpacing\":25,\"sides\":[{\"content\":{\"connectorIds\":[]},\"type\":\"ConnectorPlacement.EquallySpacedRectSide\",\"uuid\":\"288187f8-f80a-4535-8eff-6998f4e932c0\"},{\"content\":{\"connectorIds\":[\"Out1\"],\"side\":\"RIGHT\"},\"type\":\"ConnectorPlacement.EquallySpacedRectSide\",\"uuid\":\"d1e22774-cdd2-4e71-94b1-3e938d9d16f6\"},{\"content\":{\"connectorIds\":[\"In1\",\"Out2\"],\"side\":\"TOP\"},\"type\":\"ConnectorPlacement.EquallySpacedRectSide\",\"uuid\":\"890411bd-a9cd-40b1-a683-0574f0cd14d7\"}]},\"type\":\"ConnectorPlacement.EquallySpacedConnector\",\"uuid\":\"f677e6f7-ddb0-43ad-ab3a-7892dac74d79\"}],\"packageUris\":[\"http:\\/\\/schema.mathworks.com\\/mf0\\/Connector\\/19700101\"],\"version\":\"1.0\"}"
  Power Module : Subsystem
      settings: PortSchema="{\"entries\":[{\"content\":{\"headerSize\":26,\"margin\":15,\"minimumSpacing\":25,\"sides\":[{\"content\":{\"connectorIds\":[\"In1\"]},\"type\":\"ConnectorPlacement.EquallySpacedRectSide\",\"uuid\":\"410c5b0f-08b5-48c1-aeab-ad32707f18cb\"},{\"content\":{\"connectorIds\":[\"Out1\"],\"side\":\"RIGHT\"},\"type\":\"ConnectorPlacement.EquallySpacedRectSide\",\"uuid\":\"175f376c-06cb-43d8-93cf-cfe74288c6ca\"},{\"content\":{\"connectorIds\":[],\"side\":\"TOP\"},\"type\":\"ConnectorPlacement.EquallySpacedRectSide\",\"uuid\":\"49daa1ce-2b00-43ab-833d-e4aa679275fe\"}]},\"type\":\"ConnectorPlacement.EquallySpacedConnector\",\"uuid\":\"5fe6ec80-a25e-4dcf-8012-d525fb653d3d\"}],\"packageUris\":[\"http:\\/\\/schema.mathworks.com\\/mf0\\/Connector\\/19700101\"],\"version\":\"1.0\"}"
  Prop : Subsystem
      settings: PortSchema="{\"entries\":[{\"content\":{\"headerSize\":26,\"margin\":15,\"minimumSpacing\":25,\"sides\":[{\"content\":{\"connectorIds\":[\"In1\"]},\"type\":\"ConnectorPlacement.EquallySpacedRectSide\",\"uuid\":\"410c5b0f-08b5-48c1-aeab-ad32707f18cb\"},{\"content\":{\"connectorIds\":[],\"side\":\"RIGHT\"},\"type\":\"ConnectorPlacement.EquallySpacedRectSide\",\"uuid\":\"175f376c-06cb-43d8-93cf-cfe74288c6ca\"},{\"content\":{\"connectorIds\":[],\"side\":\"TOP\"},\"type\":\"ConnectorPlacement.EquallySpacedRectSide\",\"uuid\":\"49daa1ce-2b00-43ab-833d-e4aa679275fe\"}]},\"type\":\"ConnectorPlacement.EquallySpacedConnector\",\"uuid\":\"5fe6ec80-a25e-4dcf-8012-d525fb653d3d\"}],\"packageUris\":[\"http:\\/\\/schema.mathworks.com\\/mf0\\/Connector\\/19700101\"],\"version\":\"1.0\"}"
  Bus Element Out1 : Outport  VectorParamsAs1DForOutWhenUnconnected=off  PortName=EngineStatus
  Bus Element Out2 : Outport  Port=2  VectorParamsAs1DForOutWhenUnconnected=off  PortName=FuelLevel
  Bus Element Out3 : Outport  Port=3  VectorParamsAs1DForOutWhenUnconnected=off  PortName=PwrStatus
  wires:
  Fuel System/1(FuelLevel) -> Bus Element Out2/1
  Engine/3(MechConnection) -> Prop/1(Mech Connection), Power Module/1(Mech Connection)
  Power Module/1(PwrStatus) -> Bus Element Out3/1
  Bus Element In1/1 -> Engine/2(dT)
  Engine/1(EngineStatus) -> Bus Element Out1/1
  Engine/2(FuelReturn) -> Fuel System/1(FuelReturn)
  Fuel System/2(FuelSupply) -> Engine/1(FuelSupply)

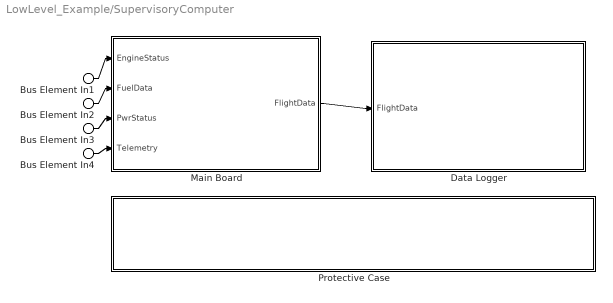
== system LowLevel_Example/SupervisoryComputer ==
  Bus Element In1 : Inport  PortName=EngineStatus
  Bus Element In2 : Inport  Port=2  PortName=FuelData
  Bus Element In3 : Inport  Port=3  PortName=PwrStatus
  Bus Element In4 : Inport  Port=4  PortName=Telemetry
  Data Logger : Subsystem
      settings: PortSchema="{\"entries\":[{\"content\":{\"headerSize\":26,\"margin\":15,\"minimumSpacing\":25,\"sides\":[{\"content\":{\"connectorIds\":[\"In1\"]},\"type\":\"ConnectorPlacement.EquallySpacedRectSide\",\"uuid\":\"410c5b0f-08b5-48c1-aeab-ad32707f18cb\"},{\"content\":{\"connectorIds\":[],\"side\":\"RIGHT\"},\"type\":\"ConnectorPlacement.EquallySpacedRectSide\",\"uuid\":\"175f376c-06cb-43d8-93cf-cfe74288c6ca\"},{\"content\":{\"connectorIds\":[],\"side\":\"TOP\"},\"type\":\"ConnectorPlacement.EquallySpacedRectSide\",\"uuid\":\"49daa1ce-2b00-43ab-833d-e4aa679275fe\"}]},\"type\":\"ConnectorPlacement.EquallySpacedConnector\",\"uuid\":\"5fe6ec80-a25e-4dcf-8012-d525fb653d3d\"}],\"packageUris\":[\"http:\\/\\/schema.mathworks.com\\/mf0\\/Connector\\/19700101\"],\"version\":\"1.0\"}"
  Main Board : Subsystem
      settings: PortSchema="{\"entries\":[{\"content\":{\"headerSize\":26,\"margin\":15,\"minimumSpacing\":25,\"sides\":[{\"content\":{\"connectorIds\":[\"In1\",\"In2\",\"In3\",\"In4\"]},\"type\":\"ConnectorPlacement.EquallySpacedRectSide\",\"uuid\":\"410c5b0f-08b5-48c1-aeab-ad32707f18cb\"},{\"content\":{\"connectorIds\":[\"Out1\"],\"side\":\"RIGHT\"},\"type\":\"ConnectorPlacement.EquallySpacedRectSide\",\"uuid\":\"175f376c-06cb-43d8-93cf-cfe74288c6ca\"},{\"content\":{\"connectorIds\":[],\"side\":\"TOP\"},\"type\":\"ConnectorPlacement.EquallySpacedRectSide\",\"uuid\":\"49daa1ce-2b00-43ab-833d-e4aa679275fe\"}]},\"type\":\"ConnectorPlacement.EquallySpacedConnector\",\"uuid\":\"5fe6ec80-a25e-4dcf-8012-d525fb653d3d\"}],\"packageUris\":[\"http:\\/\\/schema.mathworks.com\\/mf0\\/Connector\\/19700101\"],\"version\":\"1.0\"}"
  Protective Case : Subsystem
      settings: PortSchema="{\"entries\":[{\"content\":{\"headerSize\":26,\"margin\":15,\"minimumSpacing\":25,\"sides\":[{\"content\":{\"connectorIds\":[]},\"type\":\"ConnectorPlacement.EquallySpacedRectSide\",\"uuid\":\"1d3f3a23-636b-441d-85a6-b75e05b18389\"},{\"content\":{\"connectorIds\":[],\"side\":\"RIGHT\"},\"type\":\"ConnectorPlacement.EquallySpacedRectSide\",\"uuid\":\"e22d7e46-f58c-4c9d-8892-998381cd60e3\"},{\"content\":{\"connectorIds\":[],\"side\":\"TOP\"},\"type\":\"ConnectorPlacement.EquallySpacedRectSide\",\"uuid\":\"8b16ddbb-b471-4974-8372-55ce1efe9f0b\"}]},\"type\":\"ConnectorPlacement.EquallySpacedConnector\",\"uuid\":\"3aaecc83-0a24-4c0b-b096-52d61c24d002\"}],\"packageUris\":[\"http:\\/\\/schema.mathworks.com\\/mf0\\/Connector\\/19700101\"],\"version\":\"1.0\"}"
  wires:
  Bus Element In4/1 -> Main Board/4(Telemetry)
  Main Board/1(FlightData) -> Data Logger/1(FlightData)
  Bus Element In2/1 -> Main Board/2(FuelData)
  Bus Element In3/1 -> Main Board/3(PwrStatus)
  Bus Element In1/1 -> Main Board/1(EngineStatus)

== system LowLevel_Example/Airframe/Fuselage ==

== system LowLevel_Example/Airframe/LandingGear ==
  Bus Element In1 : Inport  PortName=Brake

== system LowLevel_Example/Airframe/Tail and Boom ==
  Bus Element In1 : Inport  PortName=Landing Strobe
  Bus Element In2 : Inport  Port=2  PortName=dR_dE

== system LowLevel_Example/Airframe/Wings ==
  Bus Element In1 : Inport  PortName=Navigation Lights
  Bus Element In2 : Inport  Port=2  PortName=dA_dF

== system LowLevel_Example/Flight Support Components/ADSB Module ==
  In1 : Inport  PortName=ADSBData
  ABDSB Antenna : Subsystem
      settings: PortSchema="{\"entries\":[{\"content\":{\"headerSize\":26,\"margin\":15,\"minimumSpacing\":25,\"sides\":[{\"content\":{\"connectorIds\":[]},\"type\":\"ConnectorPlacement.EquallySpacedRectSide\",\"uuid\":\"1d3f3a23-636b-441d-85a6-b75e05b18389\"},{\"content\":{\"connectorIds\":[\"In1\"],\"side\":\"RIGHT\"},\"type\":\"ConnectorPlacement.EquallySpacedRectSide\",\"uuid\":\"e22d7e46-f58c-4c9d-8892-998381cd60e3\"},{\"content\":{\"connectorIds\":[],\"side\":\"TOP\"},\"type\":\"ConnectorPlacement.EquallySpacedRectSide\",\"uuid\":\"8b16ddbb-b471-4974-8372-55ce1efe9f0b\"}]},\"type\":\"ConnectorPlacement.EquallySpacedConnector\",\"uuid\":\"3aaecc83-0a24-4c0b-b096-52d61c24d002\"}],\"packageUris\":[\"http:\\/\\/schema.mathworks.com\\/mf0\\/Connector\\/19700101\"],\"version\":\"1.0\"}"
  ADSB Board : Subsystem
      settings: PortSchema="{\"entries\":[{\"content\":{\"headerSize\":26,\"margin\":15,\"minimumSpacing\":25,\"sides\":[{\"content\":{\"connectorIds\":[]},\"type\":\"ConnectorPlacement.EquallySpacedRectSide\",\"uuid\":\"410c5b0f-08b5-48c1-aeab-ad32707f18cb\"},{\"content\":{\"connectorIds\":[\"Out1\"],\"side\":\"RIGHT\"},\"type\":\"ConnectorPlacement.EquallySpacedRectSide\",\"uuid\":\"175f376c-06cb-43d8-93cf-cfe74288c6ca\"},{\"content\":{\"connectorIds\":[],\"side\":\"TOP\"},\"type\":\"ConnectorPlacement.EquallySpacedRectSide\",\"uuid\":\"49daa1ce-2b00-43ab-833d-e4aa679275fe\"},{\"content\":{\"connectorIds\":[\"In1\"],\"side\":\"BOTTOM\"},\"type\":\"ConnectorPlacement.EquallySpacedRectSide\",\"uuid\":\"7387ed82-7e5e-434d-9bc8-2be01fbfe670\"}]},\"type\":\"ConnectorPlacement.EquallySpacedConnector\",\"uuid\":\"5fe6ec80-a25e-4dcf-8012-d525fb653d3d\"}],\"packageUris\":[\"http:\\/\\/schema.mathworks.com\\/mf0\\/Connector\\/19700101\"],\"version\":\"1.0\"}"
  wires:
  In1/1 -> ADSB Board/1(ADSBData)
  ADSB Board/1(RFSignal) -> ABDSB Antenna/1(RFSignal)

== system LowLevel_Example/Flight Support Components/GPS Module ==
  GPS Antenna : Subsystem
      settings: PortSchema="{\"entries\":[{\"content\":{\"headerSize\":26,\"margin\":15,\"minimumSpacing\":25,\"sides\":[{\"content\":{\"connectorIds\":[]},\"type\":\"ConnectorPlacement.EquallySpacedRectSide\",\"uuid\":\"1d3f3a23-636b-441d-85a6-b75e05b18389\"},{\"content\":{\"connectorIds\":[\"In1\"],\"side\":\"RIGHT\"},\"type\":\"ConnectorPlacement.EquallySpacedRectSide\",\"uuid\":\"e22d7e46-f58c-4c9d-8892-998381cd60e3\"},{\"content\":{\"connectorIds\":[],\"side\":\"TOP\"},\"type\":\"ConnectorPlacement.EquallySpacedRectSide\",\"uuid\":\"8b16ddbb-b471-4974-8372-55ce1efe9f0b\"}]},\"type\":\"ConnectorPlacement.EquallySpacedConnector\",\"uuid\":\"3aaecc83-0a24-4c0b-b096-52d61c24d002\"}],\"packageUris\":[\"http:\\/\\/schema.mathworks.com\\/mf0\\/Connector\\/19700101\"],\"version\":\"1.0\"}"
  GPS Board : Subsystem
      settings: PortSchema="{\"entries\":[{\"content\":{\"headerSize\":26,\"margin\":15,\"minimumSpacing\":25,\"sides\":[{\"content\":{\"connectorIds\":[]},\"type\":\"ConnectorPlacement.EquallySpacedRectSide\",\"uuid\":\"288187f8-f80a-4535-8eff-6998f4e932c0\"},{\"content\":{\"connectorIds\":[\"Out1\"],\"side\":\"RIGHT\"},\"type\":\"ConnectorPlacement.EquallySpacedRectSide\",\"uuid\":\"d1e22774-cdd2-4e71-94b1-3e938d9d16f6\"},{\"content\":{\"connectorIds\":[],\"side\":\"TOP\"},\"type\":\"ConnectorPlacement.EquallySpacedRectSide\",\"uuid\":\"890411bd-a9cd-40b1-a683-0574f0cd14d7\"},{\"content\":{\"connectorIds\":[\"Out2\"],\"side\":\"BOTTOM\"},\"type\":\"ConnectorPlacement.EquallySpacedRectSide\",\"uuid\":\"27348620-2e46-434a-9ea6-67f85aeb7bd2\"}]},\"type\":\"ConnectorPlacement.EquallySpacedConnector\",\"uuid\":\"f677e6f7-ddb0-43ad-ab3a-7892dac74d79\"}],\"packageUris\":[\"http:\\/\\/schema.mathworks.com\\/mf0\\/Connector\\/19700101\"],\"version\":\"1.0\"}"
  Out1 : Outport  VectorParamsAs1DForOutWhenUnconnected=off  PortName=GPSModeuleData
  wires:
  GPS Board/2(GPSData) -> Out1/1
  GPS Board/1(RFSignal) -> GPS Antenna/1(RFSignal)

== system LowLevel_Example/Flight Support Components/Pitot Tube Module ==
  Bus Element Out1 : Outport  VectorParamsAs1DForOutWhenUnconnected=off  PortName=AirData

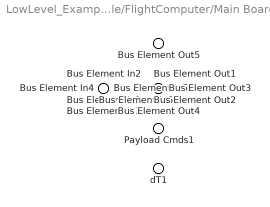
== system LowLevel_Example/FlightComputer/Main Board ==
  Bus Element In1 : Inport  PortName=AirData
  Bus Element In2 : Inport  Port=2  PortName=EngineStatus
  Bus Element In3 : Inport  Port=3  PortName=FuelLevel
  Bus Element In4 : Inport  Port=4  PortName=GPSData
  Bus Element In5 : Inport  Port=5  PortName=GS Commands
  Bus Element In6 : Inport  Port=6  PortName=PwrStatus
  Bus Element Out5 : Outport  VectorParamsAs1DForOutWhenUnconnected=off  PortName=RFSignal
  Bus Element Out1 : Outport  Port=2  VectorParamsAs1DForOutWhenUnconnected=off  PortName=ADSBData
  Bus Element Out2 : Outport  Port=3  VectorParamsAs1DForOutWhenUnconnected=off  PortName=Control Surface Cmds
  Bus Element Out3 : Outport  Port=4  VectorParamsAs1DForOutWhenUnconnected=off  PortName=Light Cmds
  Bus Element Out4 : Outport  Port=5  VectorParamsAs1DForOutWhenUnconnected=off  PortName=Telemetry
  Payload Cmds1 : Outport  Port=6  VectorParamsAs1DForOutWhenUnconnected=off  PortName=Payload Cmds
  dT1 : Outport  Port=7  VectorParamsAs1DForOutWhenUnconnected=off  PortName=dT

== system LowLevel_Example/FlightComputer/Protective Case ==

== system LowLevel_Example/FlightComputer/Telemetry Antenna ==
  Bus Element In1 : Inport  PortName=RFSignal

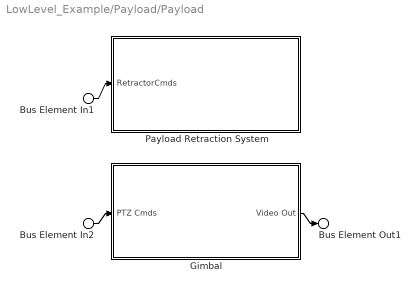
== system LowLevel_Example/Payload/Payload ==
  Bus Element In1 : Inport  PortName=operatorCmds  Element=RetractorCmds
  Bus Element In2 : Inport  PortName=operatorCmds  Element=PTZCmds
  Gimbal : Subsystem
      settings: PortSchema="{\"entries\":[{\"content\":{\"headerSize\":26,\"margin\":15,\"minimumSpacing\":25,\"sides\":[{\"content\":{\"connectorIds\":[\"In1\"]},\"type\":\"ConnectorPlacement.EquallySpacedRectSide\",\"uuid\":\"410c5b0f-08b5-48c1-aeab-ad32707f18cb\"},{\"content\":{\"connectorIds\":[\"Out1\"],\"side\":\"RIGHT\"},\"type\":\"ConnectorPlacement.EquallySpacedRectSide\",\"uuid\":\"175f376c-06cb-43d8-93cf-cfe74288c6ca\"},{\"content\":{\"connectorIds\":[],\"side\":\"TOP\"},\"type\":\"ConnectorPlacement.EquallySpacedRectSide\",\"uuid\":\"49daa1ce-2b00-43ab-833d-e4aa679275fe\"}]},\"type\":\"ConnectorPlacement.EquallySpacedConnector\",\"uuid\":\"5fe6ec80-a25e-4dcf-8012-d525fb653d3d\"}],\"packageUris\":[\"http:\\/\\/schema.mathworks.com\\/mf0\\/Connector\\/19700101\"],\"version\":\"1.0\"}"
  Payload Retraction System : Subsystem
      settings: PortSchema="{\"entries\":[{\"content\":{\"headerSize\":26,\"margin\":15,\"minimumSpacing\":25,\"sides\":[{\"content\":{\"connectorIds\":[\"In1\"]},\"type\":\"ConnectorPlacement.EquallySpacedRectSide\",\"uuid\":\"410c5b0f-08b5-48c1-aeab-ad32707f18cb\"},{\"content\":{\"connectorIds\":[],\"side\":\"RIGHT\"},\"type\":\"ConnectorPlacement.EquallySpacedRectSide\",\"uuid\":\"175f376c-06cb-43d8-93cf-cfe74288c6ca\"},{\"content\":{\"connectorIds\":[],\"side\":\"TOP\"},\"type\":\"ConnectorPlacement.EquallySpacedRectSide\",\"uuid\":\"49daa1ce-2b00-43ab-833d-e4aa679275fe\"}]},\"type\":\"ConnectorPlacement.EquallySpacedConnector\",\"uuid\":\"5fe6ec80-a25e-4dcf-8012-d525fb653d3d\"}],\"packageUris\":[\"http:\\/\\/schema.mathworks.com\\/mf0\\/Connector\\/19700101\"],\"version\":\"1.0\"}"
  Bus Element Out1 : Outport  VectorParamsAs1DForOutWhenUnconnected=off  PortName=Video Out
  wires:
  Gimbal/1(Video Out) -> Bus Element Out1/1
  Bus Element In1/1 -> Payload Retraction System/1(RetractorCmds)
  Bus Element In2/1 -> Gimbal/1(PTZ Cmds)

== system LowLevel_Example/Payload/Payload Data Link ==
  Bus Element In1 : Inport  PortName=Video In
  Bus Element Out1 : Outport  VectorParamsAs1DForOutWhenUnconnected=off  PortName=Data Link

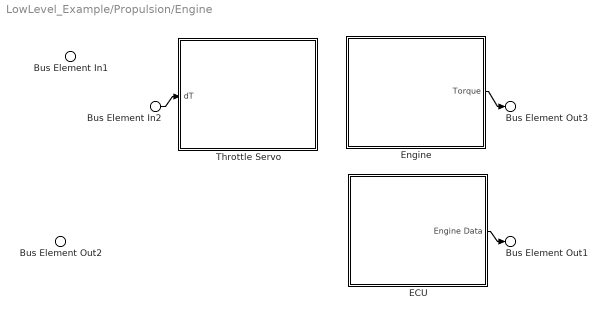
== system LowLevel_Example/Propulsion/Engine ==
  Bus Element In1 : Inport  PortName=FuelSupply
  Bus Element In2 : Inport  Port=2  PortName=dT
  ECU : Subsystem
      settings: PortSchema="{\"entries\":[{\"content\":{\"headerSize\":26,\"margin\":15,\"minimumSpacing\":25,\"sides\":[{\"content\":{\"connectorIds\":[]},\"type\":\"ConnectorPlacement.EquallySpacedRectSide\",\"uuid\":\"288187f8-f80a-4535-8eff-6998f4e932c0\"},{\"content\":{\"connectorIds\":[\"Out1\"],\"side\":\"RIGHT\"},\"type\":\"ConnectorPlacement.EquallySpacedRectSide\",\"uuid\":\"d1e22774-cdd2-4e71-94b1-3e938d9d16f6\"},{\"content\":{\"connectorIds\":[],\"side\":\"TOP\"},\"type\":\"ConnectorPlacement.EquallySpacedRectSide\",\"uuid\":\"890411bd-a9cd-40b1-a683-0574f0cd14d7\"}]},\"type\":\"ConnectorPlacement.EquallySpacedConnector\",\"uuid\":\"f677e6f7-ddb0-43ad-ab3a-7892dac74d79\"}],\"packageUris\":[\"http:\\/\\/schema.mathworks.com\\/mf0\\/Connector\\/19700101\"],\"version\":\"1.0\"}"
  Engine : Subsystem
      settings: PortSchema="{\"entries\":[{\"content\":{\"headerSize\":26,\"margin\":15,\"minimumSpacing\":25,\"sides\":[{\"content\":{\"connectorIds\":[]},\"type\":\"ConnectorPlacement.EquallySpacedRectSide\",\"uuid\":\"288187f8-f80a-4535-8eff-6998f4e932c0\"},{\"content\":{\"connectorIds\":[\"Out1\"],\"side\":\"RIGHT\"},\"type\":\"ConnectorPlacement.EquallySpacedRectSide\",\"uuid\":\"d1e22774-cdd2-4e71-94b1-3e938d9d16f6\"},{\"content\":{\"connectorIds\":[],\"side\":\"TOP\"},\"type\":\"ConnectorPlacement.EquallySpacedRectSide\",\"uuid\":\"890411bd-a9cd-40b1-a683-0574f0cd14d7\"}]},\"type\":\"ConnectorPlacement.EquallySpacedConnector\",\"uuid\":\"f677e6f7-ddb0-43ad-ab3a-7892dac74d79\"}],\"packageUris\":[\"http:\\/\\/schema.mathworks.com\\/mf0\\/Connector\\/19700101\"],\"version\":\"1.0\"}"
  Throttle Servo : Subsystem
      settings: PortSchema="{\"entries\":[{\"content\":{\"headerSize\":26,\"margin\":15,\"minimumSpacing\":25,\"sides\":[{\"content\":{\"connectorIds\":[\"In1\"]},\"type\":\"ConnectorPlacement.EquallySpacedRectSide\",\"uuid\":\"410c5b0f-08b5-48c1-aeab-ad32707f18cb\"},{\"content\":{\"connectorIds\":[],\"side\":\"RIGHT\"},\"type\":\"ConnectorPlacement.EquallySpacedRectSide\",\"uuid\":\"175f376c-06cb-43d8-93cf-cfe74288c6ca\"},{\"content\":{\"connectorIds\":[],\"side\":\"TOP\"},\"type\":\"ConnectorPlacement.EquallySpacedRectSide\",\"uuid\":\"49daa1ce-2b00-43ab-833d-e4aa679275fe\"}]},\"type\":\"ConnectorPlacement.EquallySpacedConnector\",\"uuid\":\"5fe6ec80-a25e-4dcf-8012-d525fb653d3d\"}],\"packageUris\":[\"http:\\/\\/schema.mathworks.com\\/mf0\\/Connector\\/19700101\"],\"version\":\"1.0\"}"
  Bus Element Out1 : Outport  VectorParamsAs1DForOutWhenUnconnected=off  PortName=EngineStatus
  Bus Element Out2 : Outport  Port=2  VectorParamsAs1DForOutWhenUnconnected=off  PortName=FuelReturn
  Bus Element Out3 : Outport  Port=3  VectorParamsAs1DForOutWhenUnconnected=off  PortName=MechConnection
  wires:
  ECU/1(Engine Data) -> Bus Element Out1/1
  Bus Element In2/1 -> Throttle Servo/1(dT)
  Engine/1(Torque) -> Bus Element Out3/1

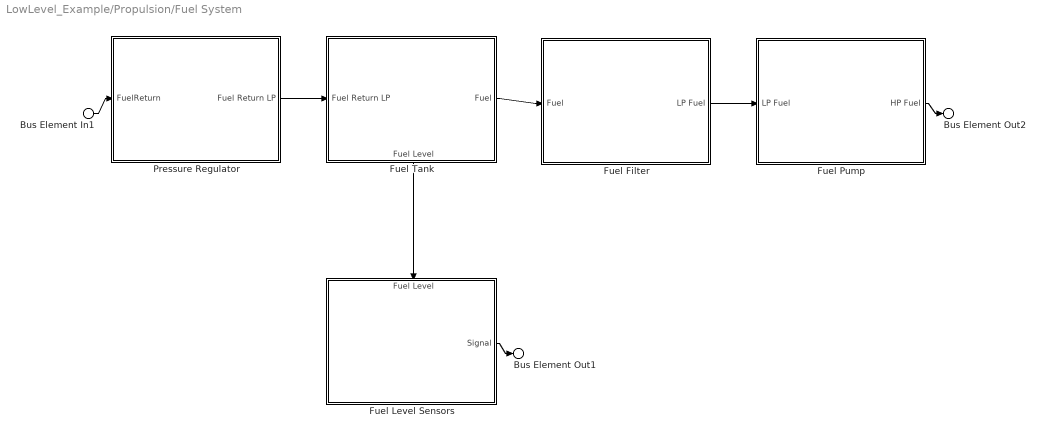
== system LowLevel_Example/Propulsion/Fuel System ==
  Bus Element In1 : Inport  PortName=FuelReturn
  Fuel Filter : Subsystem
      settings: PortSchema="{\"entries\":[{\"content\":{\"headerSize\":26,\"margin\":15,\"minimumSpacing\":25,\"sides\":[{\"content\":{\"connectorIds\":[\"In1\"]},\"type\":\"ConnectorPlacement.EquallySpacedRectSide\",\"uuid\":\"410c5b0f-08b5-48c1-aeab-ad32707f18cb\"},{\"content\":{\"connectorIds\":[\"Out1\"],\"side\":\"RIGHT\"},\"type\":\"ConnectorPlacement.EquallySpacedRectSide\",\"uuid\":\"175f376c-06cb-43d8-93cf-cfe74288c6ca\"},{\"content\":{\"connectorIds\":[],\"side\":\"TOP\"},\"type\":\"ConnectorPlacement.EquallySpacedRectSide\",\"uuid\":\"49daa1ce-2b00-43ab-833d-e4aa679275fe\"}]},\"type\":\"ConnectorPlacement.EquallySpacedConnector\",\"uuid\":\"5fe6ec80-a25e-4dcf-8012-d525fb653d3d\"}],\"packageUris\":[\"http:\\/\\/schema.mathworks.com\\/mf0\\/Connector\\/19700101\"],\"version\":\"1.0\"}"
  Fuel Level Sensors : Subsystem
      settings: PortSchema="{\"entries\":[{\"content\":{\"headerSize\":26,\"margin\":15,\"minimumSpacing\":25,\"sides\":[{\"content\":{\"connectorIds\":[]},\"type\":\"ConnectorPlacement.EquallySpacedRectSide\",\"uuid\":\"410c5b0f-08b5-48c1-aeab-ad32707f18cb\"},{\"content\":{\"connectorIds\":[\"Out1\"],\"side\":\"RIGHT\"},\"type\":\"ConnectorPlacement.EquallySpacedRectSide\",\"uuid\":\"175f376c-06cb-43d8-93cf-cfe74288c6ca\"},{\"content\":{\"connectorIds\":[\"In1\"],\"side\":\"TOP\"},\"type\":\"ConnectorPlacement.EquallySpacedRectSide\",\"uuid\":\"49daa1ce-2b00-43ab-833d-e4aa679275fe\"}]},\"type\":\"ConnectorPlacement.EquallySpacedConnector\",\"uuid\":\"5fe6ec80-a25e-4dcf-8012-d525fb653d3d\"}],\"packageUris\":[\"http:\\/\\/schema.mathworks.com\\/mf0\\/Connector\\/19700101\"],\"version\":\"1.0\"}"
  Fuel Pump : Subsystem
      settings: PortSchema="{\"entries\":[{\"content\":{\"headerSize\":26,\"margin\":15,\"minimumSpacing\":25,\"sides\":[{\"content\":{\"connectorIds\":[\"In1\"]},\"type\":\"ConnectorPlacement.EquallySpacedRectSide\",\"uuid\":\"288187f8-f80a-4535-8eff-6998f4e932c0\"},{\"content\":{\"connectorIds\":[\"Out1\"],\"side\":\"RIGHT\"},\"type\":\"ConnectorPlacement.EquallySpacedRectSide\",\"uuid\":\"d1e22774-cdd2-4e71-94b1-3e938d9d16f6\"},{\"content\":{\"connectorIds\":[],\"side\":\"TOP\"},\"type\":\"ConnectorPlacement.EquallySpacedRectSide\",\"uuid\":\"890411bd-a9cd-40b1-a683-0574f0cd14d7\"}]},\"type\":\"ConnectorPlacement.EquallySpacedConnector\",\"uuid\":\"f677e6f7-ddb0-43ad-ab3a-7892dac74d79\"}],\"packageUris\":[\"http:\\/\\/schema.mathworks.com\\/mf0\\/Connector\\/19700101\"],\"version\":\"1.0\"}"
  Fuel Tank : Subsystem
      settings: PortSchema="{\"entries\":[{\"content\":{\"headerSize\":26,\"margin\":15,\"minimumSpacing\":25,\"sides\":[{\"content\":{\"connectorIds\":[\"In1\"]},\"type\":\"ConnectorPlacement.EquallySpacedRectSide\",\"uuid\":\"288187f8-f80a-4535-8eff-6998f4e932c0\"},{\"content\":{\"connectorIds\":[\"Out1\"],\"side\":\"RIGHT\"},\"type\":\"ConnectorPlacement.EquallySpacedRectSide\",\"uuid\":\"d1e22774-cdd2-4e71-94b1-3e938d9d16f6\"},{\"content\":{\"connectorIds\":[],\"side\":\"TOP\"},\"type\":\"ConnectorPlacement.EquallySpacedRectSide\",\"uuid\":\"890411bd-a9cd-40b1-a683-0574f0cd14d7\"},{\"content\":{\"connectorIds\":[\"Out2\"],\"side\":\"BOTTOM\"},\"type\":\"ConnectorPlacement.EquallySpacedRectSide\",\"uuid\":\"9f582e97-cab8-4ca7-aff7-385988f39e0e\"}]},\"type\":\"ConnectorPlacement.EquallySpacedConnector\",\"uuid\":\"f677e6f7-ddb0-43ad-ab3a-7892dac74d79\"}],\"packageUris\":[\"http:\\/\\/schema.mathworks.com\\/mf0\\/Connector\\/19700101\"],\"version\":\"1.0\"}"
  Pressure Regulator : Subsystem
      settings: PortSchema="{\"entries\":[{\"content\":{\"headerSize\":26,\"margin\":15,\"minimumSpacing\":25,\"sides\":[{\"content\":{\"connectorIds\":[\"In1\"]},\"type\":\"ConnectorPlacement.EquallySpacedRectSide\",\"uuid\":\"288187f8-f80a-4535-8eff-6998f4e932c0\"},{\"content\":{\"connectorIds\":[\"Out1\"],\"side\":\"RIGHT\"},\"type\":\"ConnectorPlacement.EquallySpacedRectSide\",\"uuid\":\"d1e22774-cdd2-4e71-94b1-3e938d9d16f6\"},{\"content\":{\"connectorIds\":[],\"side\":\"TOP\"},\"type\":\"ConnectorPlacement.EquallySpacedRectSide\",\"uuid\":\"890411bd-a9cd-40b1-a683-0574f0cd14d7\"}]},\"type\":\"ConnectorPlacement.EquallySpacedConnector\",\"uuid\":\"f677e6f7-ddb0-43ad-ab3a-7892dac74d79\"}],\"packageUris\":[\"http:\\/\\/schema.mathworks.com\\/mf0\\/Connector\\/19700101\"],\"version\":\"1.0\"}"
  Bus Element Out1 : Outport  VectorParamsAs1DForOutWhenUnconnected=off  PortName=FuelLevel
  Bus Element Out2 : Outport  Port=2  VectorParamsAs1DForOutWhenUnconnected=off  PortName=FuelSupply
  wires:
  Fuel Tank/2(Fuel Level) -> Fuel Level Sensors/1(Fuel Level)
  Fuel Filter/1(LP Fuel) -> Fuel Pump/1(LP Fuel)
  Pressure Regulator/1(Fuel Return LP) -> Fuel Tank/1(Fuel Return LP)
  Fuel Tank/1(Fuel) -> Fuel Filter/1(Fuel)
  Bus Element In1/1 -> Pressure Regulator/1(FuelReturn)
  Fuel Level Sensors/1(Signal) -> Bus Element Out1/1
  Fuel Pump/1(HP Fuel) -> Bus Element Out2/1

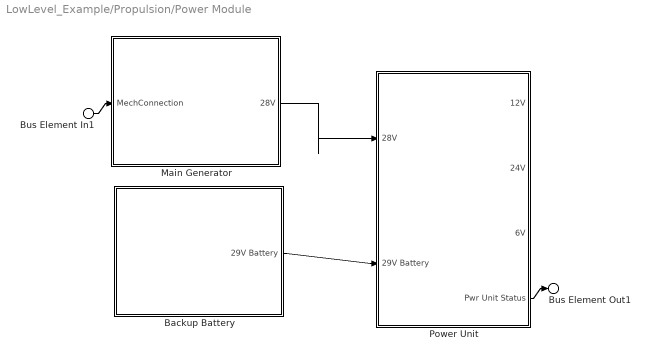
== system LowLevel_Example/Propulsion/Power Module ==
  Bus Element In1 : Inport  PortName=Mech Connection
  Backup Battery : Subsystem
      settings: PortSchema="{\"entries\":[{\"content\":{\"headerSize\":26,\"margin\":15,\"minimumSpacing\":25,\"sides\":[{\"content\":{\"connectorIds\":[]},\"type\":\"ConnectorPlacement.EquallySpacedRectSide\",\"uuid\":\"288187f8-f80a-4535-8eff-6998f4e932c0\"},{\"content\":{\"connectorIds\":[\"Out1\"],\"side\":\"RIGHT\"},\"type\":\"ConnectorPlacement.EquallySpacedRectSide\",\"uuid\":\"d1e22774-cdd2-4e71-94b1-3e938d9d16f6\"},{\"content\":{\"connectorIds\":[],\"side\":\"TOP\"},\"type\":\"ConnectorPlacement.EquallySpacedRectSide\",\"uuid\":\"890411bd-a9cd-40b1-a683-0574f0cd14d7\"}]},\"type\":\"ConnectorPlacement.EquallySpacedConnector\",\"uuid\":\"f677e6f7-ddb0-43ad-ab3a-7892dac74d79\"}],\"packageUris\":[\"http:\\/\\/schema.mathworks.com\\/mf0\\/Connector\\/19700101\"],\"version\":\"1.0\"}"
  Main Generator : Subsystem
      settings: PortSchema="{\"entries\":[{\"content\":{\"headerSize\":26,\"margin\":15,\"minimumSpacing\":25,\"sides\":[{\"content\":{\"connectorIds\":[\"In1\"]},\"type\":\"ConnectorPlacement.EquallySpacedRectSide\",\"uuid\":\"288187f8-f80a-4535-8eff-6998f4e932c0\"},{\"content\":{\"connectorIds\":[\"Out1\"],\"side\":\"RIGHT\"},\"type\":\"ConnectorPlacement.EquallySpacedRectSide\",\"uuid\":\"d1e22774-cdd2-4e71-94b1-3e938d9d16f6\"},{\"content\":{\"connectorIds\":[],\"side\":\"TOP\"},\"type\":\"ConnectorPlacement.EquallySpacedRectSide\",\"uuid\":\"890411bd-a9cd-40b1-a683-0574f0cd14d7\"}]},\"type\":\"ConnectorPlacement.EquallySpacedConnector\",\"uuid\":\"f677e6f7-ddb0-43ad-ab3a-7892dac74d79\"}],\"packageUris\":[\"http:\\/\\/schema.mathworks.com\\/mf0\\/Connector\\/19700101\"],\"version\":\"1.0\"}"
  Power Unit : Subsystem
      settings: PortSchema="{\"entries\":[{\"content\":{\"headerSize\":26,\"margin\":15,\"minimumSpacing\":25,\"sides\":[{\"content\":{\"connectorIds\":[\"In1\",\"In2\"]},\"type\":\"ConnectorPlacement.EquallySpacedRectSide\",\"uuid\":\"288187f8-f80a-4535-8eff-6998f4e932c0\"},{\"content\":{\"connectorIds\":[\"Out1\",\"Out2\",\"Out3\",\"Out4\"],\"side\":\"RIGHT\"},\"type\":\"ConnectorPlacement.EquallySpacedRectSide\",\"uuid\":\"d1e22774-cdd2-4e71-94b1-3e938d9d16f6\"},{\"content\":{\"connectorIds\":[],\"side\":\"TOP\"},\"type\":\"ConnectorPlacement.EquallySpacedRectSide\",\"uuid\":\"890411bd-a9cd-40b1-a683-0574f0cd14d7\"}]},\"type\":\"ConnectorPlacement.EquallySpacedConnector\",\"uuid\":\"f677e6f7-ddb0-43ad-ab3a-7892dac74d79\"}],\"packageUris\":[\"http:\\/\\/schema.mathworks.com\\/mf0\\/Connector\\/19700101\"],\"version\":\"1.0\"}"
  Bus Element Out1 : Outport  VectorParamsAs1DForOutWhenUnconnected=off  PortName=PwrStatus
  wires:
  Main Generator/1(28V) -> Power Unit/1(28V)
  Backup Battery/1(29V Battery) -> Power Unit/2(29V Battery)
  Bus Element In1/1 -> Main Generator/1(MechConnection)
  Power Unit/4(Pwr Unit Status) -> Bus Element Out1/1

== system LowLevel_Example/Propulsion/Prop ==
  Bus Element In1 : Inport  PortName=Mech Connection

== system LowLevel_Example/SupervisoryComputer/Data Logger ==
  Bus Element In1 : Inport  PortName=FlightData

== system LowLevel_Example/SupervisoryComputer/Main Board ==
  Bus Element In1 : Inport  PortName=EngineStatus
  Bus Element In2 : Inport  Port=2  PortName=FuelData
  Bus Element In3 : Inport  Port=3  PortName=PwrStatus
  Bus Element In4 : Inport  Port=4  PortName=Telemetry
  Bus Element Out1 : Outport  VectorParamsAs1DForOutWhenUnconnected=off  PortName=FlightData

== system LowLevel_Example/SupervisoryComputer/Protective Case ==

== system LowLevel_Example/Flight Support Components/ADSB Module/ABDSB Antenna ==
  Bus Element In1 : Inport  PortName=RFSignal

== system LowLevel_Example/Flight Support Components/ADSB Module/ADSB Board ==
  Bus Element In1 : Inport  PortName=ADSBData
  Bus Element Out1 : Outport  VectorParamsAs1DForOutWhenUnconnected=off  PortName=RFSignal

== system LowLevel_Example/Flight Support Components/GPS Module/GPS Antenna ==
  Bus Element In1 : Inport  PortName=RFSignal

== system LowLevel_Example/Flight Support Components/GPS Module/GPS Board ==
  Bus Element Out2 : Outport  VectorParamsAs1DForOutWhenUnconnected=off  PortName=RFSignal
  Bus Element Out1 : Outport  Port=2  VectorParamsAs1DForOutWhenUnconnected=off  PortName=GPSData

== system LowLevel_Example/Payload/Payload/Gimbal ==
  Bus Element In1 : Inport  PortName=PTZ Cmds
  Bus Element Out1 : Outport  VectorParamsAs1DForOutWhenUnconnected=off  PortName=Video Out

== system LowLevel_Example/Payload/Payload/Payload Retraction System ==
  Bus Element In1 : Inport  PortName=RetractorCmds
